simulink model "gm_minutiaeextraction_21821"  (R2018b)
(part 3 of 7)

  t/4845 -> concatenate37/109
  t/4846 -> concatenate37/110
  t/4847 -> concatenate37/111
  t/4848 -> concatenate37/112
  t/4849 -> concatenate37/113
  t/4850 -> concatenate37/114
  t/4851 -> concatenate37/115
  t/4852 -> concatenate37/116
  t/4853 -> concatenate37/117
  t/4854 -> concatenate37/118
  t/4855 -> concatenate37/119
  t/4856 -> concatenate37/120
  t/4857 -> concatenate37/121
  t/4858 -> concatenate37/122
  t/4859 -> concatenate37/123
  t/4860 -> concatenate37/124
  t/4861 -> concatenate37/125
  t/4862 -> concatenate37/126
  t/4863 -> concatenate37/127
  t/4864 -> concatenate37/128
  t/4865 -> concatenate38/1
  t/4866 -> concatenate38/2
  t/4867 -> concatenate38/3
  t/4868 -> concatenate38/4
  t/4869 -> concatenate38/5
  t/4870 -> concatenate38/6
  t/4871 -> concatenate38/7
  t/4872 -> concatenate38/8
  t/4873 -> concatenate38/9
  t/4874 -> concatenate38/10
  t/4875 -> concatenate38/11
  t/4876 -> concatenate38/12
  t/4877 -> concatenate38/13
  t/4878 -> concatenate38/14
  t/4879 -> concatenate38/15
  t/4880 -> concatenate38/16
  t/4881 -> concatenate38/17
  t/4882 -> concatenate38/18
  t/4883 -> concatenate38/19
  t/4884 -> concatenate38/20
  t/4885 -> concatenate38/21
  t/4886 -> concatenate38/22
  t/4887 -> concatenate38/23
  t/4888 -> concatenate38/24
  t/4889 -> concatenate38/25
  t/4890 -> concatenate38/26
  t/4891 -> concatenate38/27
  t/4892 -> concatenate38/28
  t/4893 -> concatenate38/29
  t/4894 -> concatenate38/30
  t/4895 -> concatenate38/31
  t/4896 -> concatenate38/32
  t/4897 -> concatenate38/33
  t/4898 -> concatenate38/34
  t/4899 -> concatenate38/35
  t/4900 -> concatenate38/36
  t/4901 -> concatenate38/37
  t/4902 -> concatenate38/38
  t/4903 -> concatenate38/39
  t/4904 -> concatenate38/40
  t/4905 -> concatenate38/41
  t/4906 -> concatenate38/42
  t/4907 -> concatenate38/43
  t/4908 -> concatenate38/44
  t/4909 -> concatenate38/45
  t/4910 -> concatenate38/46
  t/4911 -> concatenate38/47
  t/4912 -> concatenate38/48
  t/4913 -> concatenate38/49
  t/4914 -> concatenate38/50
  t/4915 -> concatenate38/51
  t/4916 -> concatenate38/52
  t/4917 -> concatenate38/53
  t/4918 -> concatenate38/54
  t/4919 -> concatenate38/55
  t/4920 -> concatenate38/56
  t/4921 -> concatenate38/57
  t/4922 -> concatenate38/58
  t/4923 -> concatenate38/59
  t/4924 -> concatenate38/60
  t/4925 -> concatenate38/61
  t/4926 -> concatenate38/62
  t/4927 -> concatenate38/63
  t/4928 -> concatenate38/64
  t/4929 -> concatenate38/65
  t/4930 -> concatenate38/66
  t/4931 -> concatenate38/67
  t/4932 -> concatenate38/68
  t/4933 -> concatenate38/69
  t/4934 -> concatenate38/70
  t/4935 -> concatenate38/71
  t/4936 -> concatenate38/72
  t/4937 -> concatenate38/73
  t/4938 -> concatenate38/74
  t/4939 -> concatenate38/75
  t/4940 -> concatenate38/76
  t/4941 -> concatenate38/77
  t/4942 -> concatenate38/78
  t/4943 -> concatenate38/79
  t/4944 -> concatenate38/80
  t/4945 -> concatenate38/81
  t/4946 -> concatenate38/82
  t/4947 -> concatenate38/83
  t/4948 -> concatenate38/84
  t/4949 -> concatenate38/85
  t/4950 -> concatenate38/86
  t/4951 -> concatenate38/87
  t/4952 -> concatenate38/88
  t/4953 -> concatenate38/89
  t/4954 -> concatenate38/90
  t/4955 -> concatenate38/91
  t/4956 -> concatenate38/92
  t/4957 -> concatenate38/93
  t/4958 -> concatenate38/94
  t/4959 -> concatenate38/95
  t/4960 -> concatenate38/96
  t/4961 -> concatenate38/97
  t/4962 -> concatenate38/98
  t/4963 -> concatenate38/99
  t/4964 -> concatenate38/100
  t/4965 -> concatenate38/101
  t/4966 -> concatenate38/102
  t/4967 -> concatenate38/103
  t/4968 -> concatenate38/104
  t/4969 -> concatenate38/105
  t/4970 -> concatenate38/106
  t/4971 -> concatenate38/107
  t/4972 -> concatenate38/108
  t/4973 -> concatenate38/109
  t/4974 -> concatenate38/110
  t/4975 -> concatenate38/111
  t/4976 -> concatenate38/112
  t/4977 -> concatenate38/113
  t/4978 -> concatenate38/114
  t/4979 -> concatenate38/115
  t/4980 -> concatenate38/116
  t/4981 -> concatenate38/117
  t/4982 -> concatenate38/118
  t/4983 -> concatenate38/119
  t/4984 -> concatenate38/120
  t/4985 -> concatenate38/121
  t/4986 -> concatenate38/122
  t/4987 -> concatenate38/123
  t/4988 -> concatenate38/124
  t/4989 -> concatenate38/125
  t/4990 -> concatenate38/126
  t/4991 -> concatenate38/127
  t/4992 -> concatenate38/128
  t/4993 -> concatenate39/1
  t/4994 -> concatenate39/2
  t/4995 -> concatenate39/3
  t/4996 -> concatenate39/4
  t/4997 -> concatenate39/5
  t/4998 -> concatenate39/6
  t/4999 -> concatenate39/7
  t/5000 -> concatenate39/8
  t/5001 -> concatenate39/9
  t/5002 -> concatenate39/10
  t/5003 -> concatenate39/11
  t/5004 -> concatenate39/12
  t/5005 -> concatenate39/13
  t/5006 -> concatenate39/14
  t/5007 -> concatenate39/15
  t/5008 -> concatenate39/16
  t/5009 -> concatenate39/17
  t/5010 -> concatenate39/18
  t/5011 -> concatenate39/19
  t/5012 -> concatenate39/20
  t/5013 -> concatenate39/21
  t/5014 -> concatenate39/22
  t/5015 -> concatenate39/23
  t/5016 -> concatenate39/24
  t/5017 -> concatenate39/25
  t/5018 -> concatenate39/26
  t/5019 -> concatenate39/27
  t/5020 -> concatenate39/28
  t/5021 -> concatenate39/29
  t/5022 -> concatenate39/30
  t/5023 -> concatenate39/31
  t/5024 -> concatenate39/32
  t/5025 -> concatenate39/33
  t/5026 -> concatenate39/34
  t/5027 -> concatenate39/35
  t/5028 -> concatenate39/36
  t/5029 -> concatenate39/37
  t/5030 -> concatenate39/38
  t/5031 -> concatenate39/39
  t/5032 -> concatenate39/40
  t/5033 -> concatenate39/41
  t/5034 -> concatenate39/42
  t/5035 -> concatenate39/43
  t/5036 -> concatenate39/44
  t/5037 -> concatenate39/45
  t/5038 -> concatenate39/46
  t/5039 -> concatenate39/47
  t/5040 -> concatenate39/48
  t/5041 -> concatenate39/49
  t/5042 -> concatenate39/50
  t/5043 -> concatenate39/51
  t/5044 -> concatenate39/52
  t/5045 -> concatenate39/53
  t/5046 -> concatenate39/54
  t/5047 -> concatenate39/55
  t/5048 -> concatenate39/56
  t/5049 -> concatenate39/57
  t/5050 -> concatenate39/58
  t/5051 -> concatenate39/59
  t/5052 -> concatenate39/60
  t/5053 -> concatenate39/61
  t/5054 -> concatenate39/62
  t/5055 -> concatenate39/63
  t/5056 -> concatenate39/64
  t/5057 -> concatenate39/65
  t/5058 -> concatenate39/66
  t/5059 -> concatenate39/67
  t/5060 -> concatenate39/68
  t/5061 -> concatenate39/69
  t/5062 -> concatenate39/70
  t/5063 -> concatenate39/71
  t/5064 -> concatenate39/72
  t/5065 -> concatenate39/73
  t/5066 -> concatenate39/74
  t/5067 -> concatenate39/75
  t/5068 -> concatenate39/76
  t/5069 -> concatenate39/77
  t/5070 -> concatenate39/78
  t/5071 -> concatenate39/79
  t/5072 -> concatenate39/80
  t/5073 -> concatenate39/81
  t/5074 -> concatenate39/82
  t/5075 -> concatenate39/83
  t/5076 -> concatenate39/84
  t/5077 -> concatenate39/85
  t/5078 -> concatenate39/86
  t/5079 -> concatenate39/87
  t/5080 -> concatenate39/88
  t/5081 -> concatenate39/89
  t/5082 -> concatenate39/90
  t/5083 -> concatenate39/91
  t/5084 -> concatenate39/92
  t/5085 -> concatenate39/93
  t/5086 -> concatenate39/94
  t/5087 -> concatenate39/95
  t/5088 -> concatenate39/96
  t/5089 -> concatenate39/97
  t/5090 -> concatenate39/98
  t/5091 -> concatenate39/99
  t/5092 -> concatenate39/100
  t/5093 -> concatenate39/101
  t/5094 -> concatenate39/102
  t/5095 -> concatenate39/103
  t/5096 -> concatenate39/104
  t/5097 -> concatenate39/105
  t/5098 -> concatenate39/106
  t/5099 -> concatenate39/107
  t/5100 -> concatenate39/108
  t/5101 -> concatenate39/109
  t/5102 -> concatenate39/110
  t/5103 -> concatenate39/111
  t/5104 -> concatenate39/112
  t/5105 -> concatenate39/113
  t/5106 -> concatenate39/114
  t/5107 -> concatenate39/115
  t/5108 -> concatenate39/116
  t/5109 -> concatenate39/117
  t/5110 -> concatenate39/118
  t/5111 -> concatenate39/119
  t/5112 -> concatenate39/120
  t/5113 -> concatenate39/121
  t/5114 -> concatenate39/122
  t/5115 -> concatenate39/123
  t/5116 -> concatenate39/124
  t/5117 -> concatenate39/125
  t/5118 -> concatenate39/126
  t/5119 -> concatenate39/127
  t/5120 -> concatenate39/128
  t/5121 -> concatenate40/1
  t/5122 -> concatenate40/2
  t/5123 -> concatenate40/3
  t/5124 -> concatenate40/4
  t/5125 -> concatenate40/5
  t/5126 -> concatenate40/6
  t/5127 -> concatenate40/7
  t/5128 -> concatenate40/8
  t/5129 -> concatenate40/9
  t/5130 -> concatenate40/10
  t/5131 -> concatenate40/11
  t/5132 -> concatenate40/12
  t/5133 -> concatenate40/13
  t/5134 -> concatenate40/14
  t/5135 -> concatenate40/15
  t/5136 -> concatenate40/16
  t/5137 -> concatenate40/17
  t/5138 -> concatenate40/18
  t/5139 -> concatenate40/19
  t/5140 -> concatenate40/20
  t/5141 -> concatenate40/21
  t/5142 -> concatenate40/22
  t/5143 -> concatenate40/23
  t/5144 -> concatenate40/24
  t/5145 -> concatenate40/25
  t/5146 -> concatenate40/26
  t/5147 -> concatenate40/27
  t/5148 -> concatenate40/28
  t/5149 -> concatenate40/29
  t/5150 -> concatenate40/30
  t/5151 -> concatenate40/31
  t/5152 -> concatenate40/32
  t/5153 -> concatenate40/33
  t/5154 -> concatenate40/34
  t/5155 -> concatenate40/35
  t/5156 -> concatenate40/36
  t/5157 -> concatenate40/37
  t/5158 -> concatenate40/38
  t/5159 -> concatenate40/39
  t/5160 -> concatenate40/40
  t/5161 -> concatenate40/41
  t/5162 -> concatenate40/42
  t/5163 -> concatenate40/43
  t/5164 -> concatenate40/44
  t/5165 -> concatenate40/45
  t/5166 -> concatenate40/46
  t/5167 -> concatenate40/47
  t/5168 -> concatenate40/48
  t/5169 -> concatenate40/49
  t/5170 -> concatenate40/50
  t/5171 -> concatenate40/51
  t/5172 -> concatenate40/52
  t/5173 -> concatenate40/53
  t/5174 -> concatenate40/54
  t/5175 -> concatenate40/55
  t/5176 -> concatenate40/56
  t/5177 -> concatenate40/57
  t/5178 -> concatenate40/58
  t/5179 -> concatenate40/59
  t/5180 -> concatenate40/60
  t/5181 -> concatenate40/61
  t/5182 -> concatenate40/62
  t/5183 -> concatenate40/63
  t/5184 -> concatenate40/64
  t/5185 -> concatenate40/65
  t/5186 -> concatenate40/66
  t/5187 -> concatenate40/67
  t/5188 -> concatenate40/68
  t/5189 -> concatenate40/69
  t/5190 -> concatenate40/70
  t/5191 -> concatenate40/71
  t/5192 -> concatenate40/72
  t/5193 -> concatenate40/73
  t/5194 -> concatenate40/74
  t/5195 -> concatenate40/75
  t/5196 -> concatenate40/76
  t/5197 -> concatenate40/77
  t/5198 -> concatenate40/78
  t/5199 -> concatenate40/79
  t/5200 -> concatenate40/80
  t/5201 -> concatenate40/81
  t/5202 -> concatenate40/82
  t/5203 -> concatenate40/83
  t/5204 -> concatenate40/84
  t/5205 -> concatenate40/85
  t/5206 -> concatenate40/86
  t/5207 -> concatenate40/87
  t/5208 -> concatenate40/88
  t/5209 -> concatenate40/89
  t/5210 -> concatenate40/90
  t/5211 -> concatenate40/91
  t/5212 -> concatenate40/92
  t/5213 -> concatenate40/93
  t/5214 -> concatenate40/94
  t/5215 -> concatenate40/95
  t/5216 -> concatenate40/96
  t/5217 -> concatenate40/97
  t/5218 -> concatenate40/98
  t/5219 -> concatenate40/99
  t/5220 -> concatenate40/100
  t/5221 -> concatenate40/101
  t/5222 -> concatenate40/102
  t/5223 -> concatenate40/103
  t/5224 -> concatenate40/104
  t/5225 -> concatenate40/105
  t/5226 -> concatenate40/106
  t/5227 -> concatenate40/107
  t/5228 -> concatenate40/108
  t/5229 -> concatenate40/109
  t/5230 -> concatenate40/110
  t/5231 -> concatenate40/111
  t/5232 -> concatenate40/112
  t/5233 -> concatenate40/113
  t/5234 -> concatenate40/114
  t/5235 -> concatenate40/115
  t/5236 -> concatenate40/116
  t/5237 -> concatenate40/117
  t/5238 -> concatenate40/118
  t/5239 -> concatenate40/119
  t/5240 -> concatenate40/120
  t/5241 -> concatenate40/121
  t/5242 -> concatenate40/122
  t/5243 -> concatenate40/123
  t/5244 -> concatenate40/124
  t/5245 -> concatenate40/125
  t/5246 -> concatenate40/126
  t/5247 -> concatenate40/127
  t/5248 -> concatenate40/128
  t/5249 -> concatenate41/1
  t/5250 -> concatenate41/2
  t/5251 -> concatenate41/3
  t/5252 -> concatenate41/4
  t/5253 -> concatenate41/5
  t/5254 -> concatenate41/6
  t/5255 -> concatenate41/7
  t/5256 -> concatenate41/8
  t/5257 -> concatenate41/9
  t/5258 -> concatenate41/10
  t/5259 -> concatenate41/11
  t/5260 -> concatenate41/12
  t/5261 -> concatenate41/13
  t/5262 -> concatenate41/14
  t/5263 -> concatenate41/15
  t/5264 -> concatenate41/16
  t/5265 -> concatenate41/17
  t/5266 -> concatenate41/18
  t/5267 -> concatenate41/19
  t/5268 -> concatenate41/20
  t/5269 -> concatenate41/21
  t/5270 -> concatenate41/22
  t/5271 -> concatenate41/23
  t/5272 -> concatenate41/24
  t/5273 -> concatenate41/25
  t/5274 -> concatenate41/26
  t/5275 -> concatenate41/27
  t/5276 -> concatenate41/28
  t/5277 -> concatenate41/29
  t/5278 -> concatenate41/30
  t/5279 -> concatenate41/31
  t/5280 -> concatenate41/32
  t/5281 -> concatenate41/33
  t/5282 -> concatenate41/34
  t/5283 -> concatenate41/35
  t/5284 -> concatenate41/36
  t/5285 -> concatenate41/37
  t/5286 -> concatenate41/38
  t/5287 -> concatenate41/39
  t/5288 -> concatenate41/40
  t/5289 -> concatenate41/41
  t/5290 -> concatenate41/42
  t/5291 -> concatenate41/43
  t/5292 -> concatenate41/44
  t/5293 -> concatenate41/45
  t/5294 -> concatenate41/46
  t/5295 -> concatenate41/47
  t/5296 -> concatenate41/48
  t/5297 -> concatenate41/49
  t/5298 -> concatenate41/50
  t/5299 -> concatenate41/51
  t/5300 -> concatenate41/52
  t/5301 -> concatenate41/53
  t/5302 -> concatenate41/54
  t/5303 -> concatenate41/55
  t/5304 -> concatenate41/56
  t/5305 -> concatenate41/57
  t/5306 -> concatenate41/58
  t/5307 -> concatenate41/59
  t/5308 -> concatenate41/60
  t/5309 -> concatenate41/61
  t/5310 -> concatenate41/62
  t/5311 -> concatenate41/63
  t/5312 -> concatenate41/64
  t/5313 -> concatenate41/65
  t/5314 -> concatenate41/66
  t/5315 -> concatenate41/67
  t/5316 -> concatenate41/68
  t/5317 -> concatenate41/69
  t/5318 -> concatenate41/70
  t/5319 -> concatenate41/71
  t/5320 -> concatenate41/72
  t/5321 -> concatenate41/73
  t/5322 -> concatenate41/74
  t/5323 -> concatenate41/75
  t/5324 -> concatenate41/76
  t/5325 -> concatenate41/77
  t/5326 -> concatenate41/78
  t/5327 -> concatenate41/79
  t/5328 -> concatenate41/80
  t/5329 -> concatenate41/81
  t/5330 -> concatenate41/82
  t/5331 -> concatenate41/83
  t/5332 -> concatenate41/84
  t/5333 -> concatenate41/85
  t/5334 -> concatenate41/86
  t/5335 -> concatenate41/87
  t/5336 -> concatenate41/88
  t/5337 -> concatenate41/89
  t/5338 -> concatenate41/90
  t/5339 -> concatenate41/91
  t/5340 -> concatenate41/92
  t/5341 -> concatenate41/93
  t/5342 -> concatenate41/94
  t/5343 -> concatenate41/95
  t/5344 -> concatenate41/96
  t/5345 -> concatenate41/97
  t/5346 -> concatenate41/98
  t/5347 -> concatenate41/99
  t/5348 -> concatenate41/100
  t/5349 -> concatenate41/101
  t/5350 -> concatenate41/102
  t/5351 -> concatenate41/103
  t/5352 -> concatenate41/104
  t/5353 -> concatenate41/105
  t/5354 -> concatenate41/106
  t/5355 -> concatenate41/107
  t/5356 -> concatenate41/108
  t/5357 -> concatenate41/109
  t/5358 -> concatenate41/110
  t/5359 -> concatenate41/111
  t/5360 -> concatenate41/112
  t/5361 -> concatenate41/113
  t/5362 -> concatenate41/114
  t/5363 -> concatenate41/115
  t/5364 -> concatenate41/116
  t/5365 -> concatenate41/117
  t/5366 -> concatenate41/118
  t/5367 -> concatenate41/119
  t/5368 -> concatenate41/120
  t/5369 -> concatenate41/121
  t/5370 -> concatenate41/122
  t/5371 -> concatenate41/123
  t/5372 -> concatenate41/124
  t/5373 -> concatenate41/125
  t/5374 -> concatenate41/126
  t/5375 -> concatenate41/127
  t/5376 -> concatenate41/128
  t/5377 -> concatenate42/1
  t/5378 -> concatenate42/2
  t/5379 -> concatenate42/3
  t/5380 -> concatenate42/4
  t/5381 -> concatenate42/5
  t/5382 -> concatenate42/6
  t/5383 -> concatenate42/7
  t/5384 -> concatenate42/8
  t/5385 -> concatenate42/9
  t/5386 -> concatenate42/10
  t/5387 -> concatenate42/11
  t/5388 -> concatenate42/12
  t/5389 -> concatenate42/13
  t/5390 -> concatenate42/14
  t/5391 -> concatenate42/15
  t/5392 -> concatenate42/16
  t/5393 -> concatenate42/17
  t/5394 -> concatenate42/18
  t/5395 -> concatenate42/19
  t/5396 -> concatenate42/20
  t/5397 -> concatenate42/21
  t/5398 -> concatenate42/22
  t/5399 -> concatenate42/23
  t/5400 -> concatenate42/24
  t/5401 -> concatenate42/25
  t/5402 -> concatenate42/26
  t/5403 -> concatenate42/27
  t/5404 -> concatenate42/28
  t/5405 -> concatenate42/29
  t/5406 -> concatenate42/30
  t/5407 -> concatenate42/31
  t/5408 -> concatenate42/32
  t/5409 -> concatenate42/33
  t/5410 -> concatenate42/34
  t/5411 -> concatenate42/35
  t/5412 -> concatenate42/36
  t/5413 -> concatenate42/37
  t/5414 -> concatenate42/38
  t/5415 -> concatenate42/39
  t/5416 -> concatenate42/40
  t/5417 -> concatenate42/41
  t/5418 -> concatenate42/42
  t/5419 -> concatenate42/43
  t/5420 -> concatenate42/44
  t/5421 -> concatenate42/45
  t/5422 -> concatenate42/46
  t/5423 -> concatenate42/47
  t/5424 -> concatenate42/48
  t/5425 -> concatenate42/49
  t/5426 -> concatenate42/50
  t/5427 -> concatenate42/51
  t/5428 -> concatenate42/52
  t/5429 -> concatenate42/53
  t/5430 -> concatenate42/54
  t/5431 -> concatenate42/55
  t/5432 -> concatenate42/56
  t/5433 -> concatenate42/57
  t/5434 -> concatenate42/58
  t/5435 -> concatenate42/59
  t/5436 -> concatenate42/60
  t/5437 -> concatenate42/61
  t/5438 -> concatenate42/62
  t/5439 -> concatenate42/63
  t/5440 -> concatenate42/64
  t/5441 -> concatenate42/65
  t/5442 -> concatenate42/66
  t/5443 -> concatenate42/67
  t/5444 -> concatenate42/68
  t/5445 -> concatenate42/69
  t/5446 -> concatenate42/70
  t/5447 -> concatenate42/71
  t/5448 -> concatenate42/72
  t/5449 -> concatenate42/73
  t/5450 -> concatenate42/74
  t/5451 -> concatenate42/75
  t/5452 -> concatenate42/76
  t/5453 -> concatenate42/77
  t/5454 -> concatenate42/78
  t/5455 -> concatenate42/79
  t/5456 -> concatenate42/80
  t/5457 -> concatenate42/81
  t/5458 -> concatenate42/82
  t/5459 -> concatenate42/83
  t/5460 -> concatenate42/84
  t/5461 -> concatenate42/85
  t/5462 -> concatenate42/86
  t/5463 -> concatenate42/87
  t/5464 -> concatenate42/88
  t/5465 -> concatenate42/89
  t/5466 -> concatenate42/90
  t/5467 -> concatenate42/91
  t/5468 -> concatenate42/92
  t/5469 -> concatenate42/93
  t/5470 -> concatenate42/94
  t/5471 -> concatenate42/95
  t/5472 -> concatenate42/96
  t/5473 -> concatenate42/97
  t/5474 -> concatenate42/98
  t/5475 -> concatenate42/99
  t/5476 -> concatenate42/100
  t/5477 -> concatenate42/101
  t/5478 -> concatenate42/102
  t/5479 -> concatenate42/103
  t/5480 -> concatenate42/104
  t/5481 -> concatenate42/105
  t/5482 -> concatenate42/106
  t/5483 -> concatenate42/107
  t/5484 -> concatenate42/108
  t/5485 -> concatenate42/109
  t/5486 -> concatenate42/110
  t/5487 -> concatenate42/111
  t/5488 -> concatenate42/112
  t/5489 -> concatenate42/113
  t/5490 -> concatenate42/114
  t/5491 -> concatenate42/115
  t/5492 -> concatenate42/116
  t/5493 -> concatenate42/117
  t/5494 -> concatenate42/118
  t/5495 -> concatenate42/119
  t/5496 -> concatenate42/120
  t/5497 -> concatenate42/121
  t/5498 -> concatenate42/122
  t/5499 -> concatenate42/123
  t/5500 -> concatenate42/124
  t/5501 -> concatenate42/125
  t/5502 -> concatenate42/126
  t/5503 -> concatenate42/127
  t/5504 -> concatenate42/128
  t/5505 -> concatenate43/1
  t/5506 -> concatenate43/2
  t/5507 -> concatenate43/3
  t/5508 -> concatenate43/4
  t/5509 -> concatenate43/5
  t/5510 -> concatenate43/6
  t/5511 -> concatenate43/7
  t/5512 -> concatenate43/8
  t/5513 -> concatenate43/9
  t/5514 -> concatenate43/10
  t/5515 -> concatenate43/11
  t/5516 -> concatenate43/12
  t/5517 -> concatenate43/13
  t/5518 -> concatenate43/14
  t/5519 -> concatenate43/15
  t/5520 -> concatenate43/16
  t/5521 -> concatenate43/17
  t/5522 -> concatenate43/18
  t/5523 -> concatenate43/19
  t/5524 -> concatenate43/20
  t/5525 -> concatenate43/21
  t/5526 -> concatenate43/22
  t/5527 -> concatenate43/23
  t/5528 -> concatenate43/24
  t/5529 -> concatenate43/25
  t/5530 -> concatenate43/26
  t/5531 -> concatenate43/27
  t/5532 -> concatenate43/28
  t/5533 -> concatenate43/29
  t/5534 -> concatenate43/30
  t/5535 -> concatenate43/31
  t/5536 -> concatenate43/32
  t/5537 -> concatenate43/33
  t/5538 -> concatenate43/34
  t/5539 -> concatenate43/35
  t/5540 -> concatenate43/36
  t/5541 -> concatenate43/37
  t/5542 -> concatenate43/38
  t/5543 -> concatenate43/39
  t/5544 -> concatenate43/40
  t/5545 -> concatenate43/41
  t/5546 -> concatenate43/42
  t/5547 -> concatenate43/43
  t/5548 -> concatenate43/44
  t/5549 -> concatenate43/45
  t/5550 -> concatenate43/46
  t/5551 -> concatenate43/47
  t/5552 -> concatenate43/48
  t/5553 -> concatenate43/49
  t/5554 -> concatenate43/50
  t/5555 -> concatenate43/51
  t/5556 -> concatenate43/52
  t/5557 -> concatenate43/53
  t/5558 -> concatenate43/54
  t/5559 -> concatenate43/55
  t/5560 -> concatenate43/56
  t/5561 -> concatenate43/57
  t/5562 -> concatenate43/58
  t/5563 -> concatenate43/59
  t/5564 -> concatenate43/60
  t/5565 -> concatenate43/61
  t/5566 -> concatenate43/62
  t/5567 -> concatenate43/63
  t/5568 -> concatenate43/64
  t/5569 -> concatenate43/65
  t/5570 -> concatenate43/66
  t/5571 -> concatenate43/67
  t/5572 -> concatenate43/68
  t/5573 -> concatenate43/69
  t/5574 -> concatenate43/70
  t/5575 -> concatenate43/71
  t/5576 -> concatenate43/72
  t/5577 -> concatenate43/73
  t/5578 -> concatenate43/74
  t/5579 -> concatenate43/75
  t/5580 -> concatenate43/76
  t/5581 -> concatenate43/77
  t/5582 -> concatenate43/78
  t/5583 -> concatenate43/79
  t/5584 -> concatenate43/80
  t/5585 -> concatenate43/81
  t/5586 -> concatenate43/82
  t/5587 -> concatenate43/83
  t/5588 -> concatenate43/84
  t/5589 -> concatenate43/85
  t/5590 -> concatenate43/86
  t/5591 -> concatenate43/87
  t/5592 -> concatenate43/88
  t/5593 -> concatenate43/89
  t/5594 -> concatenate43/90
  t/5595 -> concatenate43/91
  t/5596 -> concatenate43/92
  t/5597 -> concatenate43/93
  t/5598 -> concatenate43/94
  t/5599 -> concatenate43/95
  t/5600 -> concatenate43/96
  t/5601 -> concatenate43/97
  t/5602 -> concatenate43/98
  t/5603 -> concatenate43/99
  t/5604 -> concatenate43/100
  t/5605 -> concatenate43/101
  t/5606 -> concatenate43/102
  t/5607 -> concatenate43/103
  t/5608 -> concatenate43/104
  t/5609 -> concatenate43/105
  t/5610 -> concatenate43/106
  t/5611 -> concatenate43/107
  t/5612 -> concatenate43/108
  t/5613 -> concatenate43/109
  t/5614 -> concatenate43/110
  t/5615 -> concatenate43/111
  t/5616 -> concatenate43/112
  t/5617 -> concatenate43/113
  t/5618 -> concatenate43/114
  t/5619 -> concatenate43/115
  t/5620 -> concatenate43/116
  t/5621 -> concatenate43/117
  t/5622 -> concatenate43/118
  t/5623 -> concatenate43/119
  t/5624 -> concatenate43/120
  t/5625 -> concatenate43/121
  t/5626 -> concatenate43/122
  t/5627 -> concatenate43/123
  t/5628 -> concatenate43/124
  t/5629 -> concatenate43/125
  t/5630 -> concatenate43/126
  t/5631 -> concatenate43/127
  t/5632 -> concatenate43/128
  t/5633 -> concatenate44/1
  t/5634 -> concatenate44/2
  t/5635 -> concatenate44/3
  t/5636 -> concatenate44/4
  t/5637 -> concatenate44/5
  t/5638 -> concatenate44/6
  t/5639 -> concatenate44/7
  t/5640 -> concatenate44/8
  t/5641 -> concatenate44/9
  t/5642 -> concatenate44/10
  t/5643 -> concatenate44/11
  t/5644 -> concatenate44/12
  t/5645 -> concatenate44/13
  t/5646 -> concatenate44/14
  t/5647 -> concatenate44/15
  t/5648 -> concatenate44/16
  t/5649 -> concatenate44/17
  t/5650 -> concatenate44/18
  t/5651 -> concatenate44/19
  t/5652 -> concatenate44/20
  t/5653 -> concatenate44/21
  t/5654 -> concatenate44/22
  t/5655 -> concatenate44/23
  t/5656 -> concatenate44/24
  t/5657 -> concatenate44/25
  t/5658 -> concatenate44/26
  t/5659 -> concatenate44/27
  t/5660 -> concatenate44/28
  t/5661 -> concatenate44/29
  t/5662 -> concatenate44/30
  t/5663 -> concatenate44/31
  t/5664 -> concatenate44/32
  t/5665 -> concatenate44/33
  t/5666 -> concatenate44/34
  t/5667 -> concatenate44/35
  t/5668 -> concatenate44/36
  t/5669 -> concatenate44/37
  t/5670 -> concatenate44/38
  t/5671 -> concatenate44/39
  t/5672 -> concatenate44/40
  t/5673 -> concatenate44/41
  t/5674 -> concatenate44/42
  t/5675 -> concatenate44/43
  t/5676 -> concatenate44/44
  t/5677 -> concatenate44/45
  t/5678 -> concatenate44/46
  t/5679 -> concatenate44/47
  t/5680 -> concatenate44/48
  t/5681 -> concatenate44/49
  t/5682 -> concatenate44/50
  t/5683 -> concatenate44/51
  t/5684 -> concatenate44/52
  t/5685 -> concatenate44/53
  t/5686 -> concatenate44/54
  t/5687 -> concatenate44/55
  t/5688 -> concatenate44/56
  t/5689 -> concatenate44/57
  t/5690 -> concatenate44/58
  t/5691 -> concatenate44/59
  t/5692 -> concatenate44/60
  t/5693 -> concatenate44/61
  t/5694 -> concatenate44/62
  t/5695 -> concatenate44/63
  t/5696 -> concatenate44/64
  t/5697 -> concatenate44/65
  t/5698 -> concatenate44/66
  t/5699 -> concatenate44/67
  t/5700 -> concatenate44/68
  t/5701 -> concatenate44/69
  t/5702 -> concatenate44/70
  t/5703 -> concatenate44/71
  t/5704 -> concatenate44/72
  t/5705 -> concatenate44/73
  t/5706 -> concatenate44/74
  t/5707 -> concatenate44/75
  t/5708 -> concatenate44/76
  t/5709 -> concatenate44/77
  t/5710 -> concatenate44/78
  t/5711 -> concatenate44/79
  t/5712 -> concatenate44/80
  t/5713 -> concatenate44/81
  t/5714 -> concatenate44/82
  t/5715 -> concatenate44/83
  t/5716 -> concatenate44/84
  t/5717 -> concatenate44/85
  t/5718 -> concatenate44/86
  t/5719 -> concatenate44/87
  t/5720 -> concatenate44/88
  t/5721 -> concatenate44/89
  t/5722 -> concatenate44/90
  t/5723 -> concatenate44/91
  t/5724 -> concatenate44/92
  t/5725 -> concatenate44/93
  t/5726 -> concatenate44/94
  t/5727 -> concatenate44/95
  t/5728 -> concatenate44/96
  t/5729 -> concatenate44/97
  t/5730 -> concatenate44/98
  t/5731 -> concatenate44/99
  t/5732 -> concatenate44/100
  t/5733 -> concatenate44/101
  t/5734 -> concatenate44/102
  t/5735 -> concatenate44/103
  t/5736 -> concatenate44/104
  t/5737 -> concatenate44/105
  t/5738 -> concatenate44/106
  t/5739 -> concatenate44/107
  t/5740 -> concatenate44/108
  t/5741 -> concatenate44/109
  t/5742 -> concatenate44/110
  t/5743 -> concatenate44/111
  t/5744 -> concatenate44/112
  t/5745 -> concatenate44/113
  t/5746 -> concatenate44/114
  t/5747 -> concatenate44/115
  t/5748 -> concatenate44/116
  t/5749 -> concatenate44/117
  t/5750 -> concatenate44/118
  t/5751 -> concatenate44/119
  t/5752 -> concatenate44/120
  t/5753 -> concatenate44/121
  t/5754 -> concatenate44/122
  t/5755 -> concatenate44/123
  t/5756 -> concatenate44/124
  t/5757 -> concatenate44/125
  t/5758 -> concatenate44/126
  t/5759 -> concatenate44/127
  t/5760 -> concatenate44/128
  t/5761 -> concatenate45/1
  t/5762 -> concatenate45/2
  t/5763 -> concatenate45/3
  t/5764 -> concatenate45/4
  t/5765 -> concatenate45/5
  t/5766 -> concatenate45/6
  t/5767 -> concatenate45/7
  t/5768 -> concatenate45/8
  t/5769 -> concatenate45/9
  t/5770 -> concatenate45/10
  t/5771 -> concatenate45/11
  t/5772 -> concatenate45/12
  t/5773 -> concatenate45/13
  t/5774 -> concatenate45/14
  t/5775 -> concatenate45/15
  t/5776 -> concatenate45/16
  t/5777 -> concatenate45/17
  t/5778 -> concatenate45/18
  t/5779 -> concatenate45/19
  t/5780 -> concatenate45/20
  t/5781 -> concatenate45/21
  t/5782 -> concatenate45/22
  t/5783 -> concatenate45/23
  t/5784 -> concatenate45/24
  t/5785 -> concatenate45/25
  t/5786 -> concatenate45/26
  t/5787 -> concatenate45/27
  t/5788 -> concatenate45/28
  t/5789 -> concatenate45/29
  t/5790 -> concatenate45/30
  t/5791 -> concatenate45/31
  t/5792 -> concatenate45/32
  t/5793 -> concatenate45/33
  t/5794 -> concatenate45/34
  t/5795 -> concatenate45/35
  t/5796 -> concatenate45/36
  t/5797 -> concatenate45/37
  t/5798 -> concatenate45/38
  t/5799 -> concatenate45/39
  t/5800 -> concatenate45/40
  t/5801 -> concatenate45/41
  t/5802 -> concatenate45/42
  t/5803 -> concatenate45/43
  t/5804 -> concatenate45/44
  t/5805 -> concatenate45/45
  t/5806 -> concatenate45/46
  t/5807 -> concatenate45/47
  t/5808 -> concatenate45/48
  t/5809 -> concatenate45/49
  t/5810 -> concatenate45/50
  t/5811 -> concatenate45/51
  t/5812 -> concatenate45/52
  t/5813 -> concatenate45/53
  t/5814 -> concatenate45/54
  t/5815 -> concatenate45/55
  t/5816 -> concatenate45/56
  t/5817 -> concatenate45/57
  t/5818 -> concatenate45/58
  t/5819 -> concatenate45/59
  t/5820 -> concatenate45/60
  t/5821 -> concatenate45/61
  t/5822 -> concatenate45/62
  t/5823 -> concatenate45/63
  t/5824 -> concatenate45/64
  t/5825 -> concatenate45/65
  t/5826 -> concatenate45/66
  t/5827 -> concatenate45/67
  t/5828 -> concatenate45/68
  t/5829 -> concatenate45/69
  t/5830 -> concatenate45/70
  t/5831 -> concatenate45/71
  t/5832 -> concatenate45/72
  t/5833 -> concatenate45/73
  t/5834 -> concatenate45/74
  t/5835 -> concatenate45/75
  t/5836 -> concatenate45/76
  t/5837 -> concatenate45/77
  t/5838 -> concatenate45/78
  t/5839 -> concatenate45/79
  t/5840 -> concatenate45/80
  t/5841 -> concatenate45/81
  t/5842 -> concatenate45/82
  t/5843 -> concatenate45/83
  t/5844 -> concatenate45/84
  t/5845 -> concatenate45/85
  t/5846 -> concatenate45/86
  t/5847 -> concatenate45/87
  t/5848 -> concatenate45/88
  t/5849 -> concatenate45/89
  t/5850 -> concatenate45/90
  t/5851 -> concatenate45/91
  t/5852 -> concatenate45/92
  t/5853 -> concatenate45/93
  t/5854 -> concatenate45/94
  t/5855 -> concatenate45/95
  t/5856 -> concatenate45/96
  t/5857 -> concatenate45/97
  t/5858 -> concatenate45/98
  t/5859 -> concatenate45/99
  t/5860 -> concatenate45/100
  t/5861 -> concatenate45/101
  t/5862 -> concatenate45/102
  t/5863 -> concatenate45/103
  t/5864 -> concatenate45/104
  t/5865 -> concatenate45/105
  t/5866 -> concatenate45/106
  t/5867 -> concatenate45/107
  t/5868 -> concatenate45/108
  t/5869 -> concatenate45/109
  t/5870 -> concatenate45/110
  t/5871 -> concatenate45/111
  t/5872 -> concatenate45/112
  t/5873 -> concatenate45/113
  t/5874 -> concatenate45/114
  t/5875 -> concatenate45/115
  t/5876 -> concatenate45/116
  t/5877 -> concatenate45/117
  t/5878 -> concatenate45/118
  t/5879 -> concatenate45/119
  t/5880 -> concatenate45/120
  t/5881 -> concatenate45/121
  t/5882 -> concatenate45/122
  t/5883 -> concatenate45/123
  t/5884 -> concatenate45/124
  t/5885 -> concatenate45/125
  t/5886 -> concatenate45/126
  t/5887 -> concatenate45/127
  t/5888 -> concatenate45/128
  t/5889 -> concatenate46/1
  t/5890 -> concatenate46/2
  t/5891 -> concatenate46/3
  t/5892 -> concatenate46/4
  t/5893 -> concatenate46/5
  t/5894 -> concatenate46/6
  t/5895 -> concatenate46/7
  t/5896 -> concatenate46/8
  t/5897 -> concatenate46/9
  t/5898 -> concatenate46/10
  t/5899 -> concatenate46/11
  t/5900 -> concatenate46/12
  t/5901 -> concatenate46/13
  t/5902 -> concatenate46/14
  t/5903 -> concatenate46/15
  t/5904 -> concatenate46/16
  t/5905 -> concatenate46/17
  t/5906 -> concatenate46/18
  t/5907 -> concatenate46/19
  t/5908 -> concatenate46/20
  t/5909 -> concatenate46/21
  t/5910 -> concatenate46/22
  t/5911 -> concatenate46/23
  t/5912 -> concatenate46/24
  t/5913 -> concatenate46/25
  t/5914 -> concatenate46/26
  t/5915 -> concatenate46/27
  t/5916 -> concatenate46/28
  t/5917 -> concatenate46/29
  t/5918 -> concatenate46/30
  t/5919 -> concatenate46/31
  t/5920 -> concatenate46/32
  t/5921 -> concatenate46/33
  t/5922 -> concatenate46/34
  t/5923 -> concatenate46/35
  t/5924 -> concatenate46/36
  t/5925 -> concatenate46/37
  t/5926 -> concatenate46/38
  t/5927 -> concatenate46/39
  t/5928 -> concatenate46/40
  t/5929 -> concatenate46/41
  t/5930 -> concatenate46/42
  t/5931 -> concatenate46/43
  t/5932 -> concatenate46/44
  t/5933 -> concatenate46/45
  t/5934 -> concatenate46/46
  t/5935 -> concatenate46/47
  t/5936 -> concatenate46/48
  t/5937 -> concatenate46/49
  t/5938 -> concatenate46/50
  t/5939 -> concatenate46/51
  t/5940 -> concatenate46/52
  t/5941 -> concatenate46/53
  t/5942 -> concatenate46/54
  t/5943 -> concatenate46/55
  t/5944 -> concatenate46/56
  t/5945 -> concatenate46/57
  t/5946 -> concatenate46/58
  t/5947 -> concatenate46/59
  t/5948 -> concatenate46/60
  t/5949 -> concatenate46/61
  t/5950 -> concatenate46/62
  t/5951 -> concatenate46/63
  t/5952 -> concatenate46/64
  t/5953 -> concatenate46/65
  t/5954 -> concatenate46/66
  t/5955 -> concatenate46/67
  t/5956 -> concatenate46/68
  t/5957 -> concatenate46/69
  t/5958 -> concatenate46/70
  t/5959 -> concatenate46/71
  t/5960 -> concatenate46/72
  t/5961 -> concatenate46/73
  t/5962 -> concatenate46/74
  t/5963 -> concatenate46/75
  t/5964 -> concatenate46/76
  t/5965 -> concatenate46/77
  t/5966 -> concatenate46/78
  t/5967 -> concatenate46/79
  t/5968 -> concatenate46/80
  t/5969 -> concatenate46/81
  t/5970 -> concatenate46/82
  t/5971 -> concatenate46/83
  t/5972 -> concatenate46/84
  t/5973 -> concatenate46/85
  t/5974 -> concatenate46/86
  t/5975 -> concatenate46/87
  t/5976 -> concatenate46/88
  t/5977 -> concatenate46/89
  t/5978 -> concatenate46/90
  t/5979 -> concatenate46/91
  t/5980 -> concatenate46/92
  t/5981 -> concatenate46/93
  t/5982 -> concatenate46/94
  t/5983 -> concatenate46/95
  t/5984 -> concatenate46/96
  t/5985 -> concatenate46/97
  t/5986 -> concatenate46/98
  t/5987 -> concatenate46/99
  t/5988 -> concatenate46/100
  t/5989 -> concatenate46/101
  t/5990 -> concatenate46/102
  t/5991 -> concatenate46/103
  t/5992 -> concatenate46/104
  t/5993 -> concatenate46/105
  t/5994 -> concatenate46/106
  t/5995 -> concatenate46/107
  t/5996 -> concatenate46/108
  t/5997 -> concatenate46/109
  t/5998 -> concatenate46/110
  t/5999 -> concatenate46/111
  t/6000 -> concatenate46/112
  t/6001 -> concatenate46/113
  t/6002 -> concatenate46/114
  t/6003 -> concatenate46/115
  t/6004 -> concatenate46/116
  t/6005 -> concatenate46/117
  t/6006 -> concatenate46/118
  t/6007 -> concatenate46/119
  t/6008 -> concatenate46/120
  t/6009 -> concatenate46/121
  t/6010 -> concatenate46/122
  t/6011 -> concatenate46/123
  t/6012 -> concatenate46/124
  t/6013 -> concatenate46/125
  t/6014 -> concatenate46/126
  t/6015 -> concatenate46/127
  t/6016 -> concatenate46/128
  t/6017 -> concatenate47/1
  t/6018 -> concatenate47/2
  t/6019 -> concatenate47/3
  t/6020 -> concatenate47/4
  t/6021 -> concatenate47/5
  t/6022 -> concatenate47/6
  t/6023 -> concatenate47/7
  t/6024 -> concatenate47/8
  t/6025 -> concatenate47/9
  t/6026 -> concatenate47/10
  t/6027 -> concatenate47/11
  t/6028 -> concatenate47/12
  t/6029 -> concatenate47/13
  t/6030 -> concatenate47/14
  t/6031 -> concatenate47/15
  t/6032 -> concatenate47/16
  t/6033 -> concatenate47/17
  t/6034 -> concatenate47/18
  t/6035 -> concatenate47/19
  t/6036 -> concatenate47/20
  t/6037 -> concatenate47/21
  t/6038 -> concatenate47/22
  t/6039 -> concatenate47/23
  t/6040 -> concatenate47/24
  t/6041 -> concatenate47/25
  t/6042 -> concatenate47/26
  t/6043 -> concatenate47/27
  t/6044 -> concatenate47/28
  t/6045 -> concatenate47/29
  t/6046 -> concatenate47/30
  t/6047 -> concatenate47/31
  t/6048 -> concatenate47/32
  t/6049 -> concatenate47/33
  t/6050 -> concatenate47/34
  t/6051 -> concatenate47/35
  t/6052 -> concatenate47/36
  t/6053 -> concatenate47/37
  t/6054 -> concatenate47/38
  t/6055 -> concatenate47/39
  t/6056 -> concatenate47/40
  t/6057 -> concatenate47/41
  t/6058 -> concatenate47/42
  t/6059 -> concatenate47/43
  t/6060 -> concatenate47/44
  t/6061 -> concatenate47/45
  t/6062 -> concatenate47/46
  t/6063 -> concatenate47/47
  t/6064 -> concatenate47/48
  t/6065 -> concatenate47/49
  t/6066 -> concatenate47/50
  t/6067 -> concatenate47/51
  t/6068 -> concatenate47/52
  t/6069 -> concatenate47/53
  t/6070 -> concatenate47/54
  t/6071 -> concatenate47/55
  t/6072 -> concatenate47/56
  t/6073 -> concatenate47/57
  t/6074 -> concatenate47/58
  t/6075 -> concatenate47/59
  t/6076 -> concatenate47/60
  t/6077 -> concatenate47/61
  t/6078 -> concatenate47/62
  t/6079 -> concatenate47/63
  t/6080 -> concatenate47/64
  t/6081 -> concatenate47/65
  t/6082 -> concatenate47/66
  t/6083 -> concatenate47/67
  t/6084 -> concatenate47/68
  t/6085 -> concatenate47/69
  t/6086 -> concatenate47/70
  t/6087 -> concatenate47/71
  t/6088 -> concatenate47/72
  t/6089 -> concatenate47/73
  t/6090 -> concatenate47/74
  t/6091 -> concatenate47/75
  t/6092 -> concatenate47/76
  t/6093 -> concatenate47/77
  t/6094 -> concatenate47/78
  t/6095 -> concatenate47/79
  t/6096 -> concatenate47/80
  t/6097 -> concatenate47/81
  t/6098 -> concatenate47/82
  t/6099 -> concatenate47/83
  t/6100 -> concatenate47/84
  t/6101 -> concatenate47/85
  t/6102 -> concatenate47/86
  t/6103 -> concatenate47/87
  t/6104 -> concatenate47/88
  t/6105 -> concatenate47/89
  t/6106 -> concatenate47/90
  t/6107 -> concatenate47/91
  t/6108 -> concatenate47/92
  t/6109 -> concatenate47/93
  t/6110 -> concatenate47/94
  t/6111 -> concatenate47/95
  t/6112 -> concatenate47/96
  t/6113 -> concatenate47/97
  t/6114 -> concatenate47/98
  t/6115 -> concatenate47/99
  t/6116 -> concatenate47/100
  t/6117 -> concatenate47/101
  t/6118 -> concatenate47/102
  t/6119 -> concatenate47/103
  t/6120 -> concatenate47/104
  t/6121 -> concatenate47/105
  t/6122 -> concatenate47/106
  t/6123 -> concatenate47/107
  t/6124 -> concatenate47/108
  t/6125 -> concatenate47/109
  t/6126 -> concatenate47/110
  t/6127 -> concatenate47/111
  t/6128 -> concatenate47/112
  t/6129 -> concatenate47/113
  t/6130 -> concatenate47/114
  t/6131 -> concatenate47/115
  t/6132 -> concatenate47/116
  t/6133 -> concatenate47/117
  t/6134 -> concatenate47/118
  t/6135 -> concatenate47/119
  t/6136 -> concatenate47/120
  t/6137 -> concatenate47/121
  t/6138 -> concatenate47/122
  t/6139 -> concatenate47/123
  t/6140 -> concatenate47/124
  t/6141 -> concatenate47/125
  t/6142 -> concatenate47/126
  t/6143 -> concatenate47/127
  t/6144 -> concatenate47/128
  t/6145 -> concatenate48/1
  t/6146 -> concatenate48/2
  t/6147 -> concatenate48/3
  t/6148 -> concatenate48/4
  t/6149 -> concatenate48/5
  t/6150 -> concatenate48/6
  t/6151 -> concatenate48/7
  t/6152 -> concatenate48/8
  t/6153 -> concatenate48/9
  t/6154 -> concatenate48/10
  t/6155 -> concatenate48/11
  t/6156 -> concatenate48/12
  t/6157 -> concatenate48/13
  t/6158 -> concatenate48/14
  t/6159 -> concatenate48/15
  t/6160 -> concatenate48/16
  t/6161 -> concatenate48/17
  t/6162 -> concatenate48/18
  t/6163 -> concatenate48/19
  t/6164 -> concatenate48/20
  t/6165 -> concatenate48/21
  t/6166 -> concatenate48/22
  t/6167 -> concatenate48/23
  t/6168 -> concatenate48/24
  t/6169 -> concatenate48/25
  t/6170 -> concatenate48/26
  t/6171 -> concatenate48/27
  t/6172 -> concatenate48/28
  t/6173 -> concatenate48/29
  t/6174 -> concatenate48/30
  t/6175 -> concatenate48/31
  t/6176 -> concatenate48/32
  t/6177 -> concatenate48/33
  t/6178 -> concatenate48/34
  t/6179 -> concatenate48/35
  t/6180 -> concatenate48/36
  t/6181 -> concatenate48/37
  t/6182 -> concatenate48/38
  t/6183 -> concatenate48/39
  t/6184 -> concatenate48/40
  t/6185 -> concatenate48/41
  t/6186 -> concatenate48/42
  t/6187 -> concatenate48/43
  t/6188 -> concatenate48/44
  t/6189 -> concatenate48/45
  t/6190 -> concatenate48/46
  t/6191 -> concatenate48/47
  t/6192 -> concatenate48/48
  t/6193 -> concatenate48/49
  t/6194 -> concatenate48/50
  t/6195 -> concatenate48/51
  t/6196 -> concatenate48/52
  t/6197 -> concatenate48/53
  t/6198 -> concatenate48/54
  t/6199 -> concatenate48/55
  t/6200 -> concatenate48/56
  t/6201 -> concatenate48/57
  t/6202 -> concatenate48/58
  t/6203 -> concatenate48/59
  t/6204 -> concatenate48/60
  t/6205 -> concatenate48/61
  t/6206 -> concatenate48/62
  t/6207 -> concatenate48/63
  t/6208 -> concatenate48/64
  t/6209 -> concatenate48/65
  t/6210 -> concatenate48/66
  t/6211 -> concatenate48/67
  t/6212 -> concatenate48/68
  t/6213 -> concatenate48/69
  t/6214 -> concatenate48/70
  t/6215 -> concatenate48/71
  t/6216 -> concatenate48/72
  t/6217 -> concatenate48/73
  t/6218 -> concatenate48/74
  t/6219 -> concatenate48/75
  t/6220 -> concatenate48/76
  t/6221 -> concatenate48/77
  t/6222 -> concatenate48/78
  t/6223 -> concatenate48/79
  t/6224 -> concatenate48/80
  t/6225 -> concatenate48/81
  t/6226 -> concatenate48/82
  t/6227 -> concatenate48/83
  t/6228 -> concatenate48/84
  t/6229 -> concatenate48/85
  t/6230 -> concatenate48/86
  t/6231 -> concatenate48/87
  t/6232 -> concatenate48/88
  t/6233 -> concatenate48/89
  t/6234 -> concatenate48/90
  t/6235 -> concatenate48/91
  t/6236 -> concatenate48/92
  t/6237 -> concatenate48/93
  t/6238 -> concatenate48/94
  t/6239 -> concatenate48/95
  t/6240 -> concatenate48/96
  t/6241 -> concatenate48/97
  t/6242 -> concatenate48/98
  t/6243 -> concatenate48/99
  t/6244 -> concatenate48/100
  t/6245 -> concatenate48/101
  t/6246 -> concatenate48/102
  t/6247 -> concatenate48/103
  t/6248 -> concatenate48/104
  t/6249 -> concatenate48/105
  t/6250 -> concatenate48/106
  t/6251 -> concatenate48/107
  t/6252 -> concatenate48/108
  t/6253 -> concatenate48/109
  t/6254 -> concatenate48/110
  t/6255 -> concatenate48/111
  t/6256 -> concatenate48/112
  t/6257 -> concatenate48/113
  t/6258 -> concatenate48/114
  t/6259 -> concatenate48/115
  t/6260 -> concatenate48/116
  t/6261 -> concatenate48/117
  t/6262 -> concatenate48/118
  t/6263 -> concatenate48/119
  t/6264 -> concatenate48/120
  t/6265 -> concatenate48/121
  t/6266 -> concatenate48/122
  t/6267 -> concatenate48/123
  t/6268 -> concatenate48/124
  t/6269 -> concatenate48/125
  t/6270 -> concatenate48/126
  t/6271 -> concatenate48/127
  t/6272 -> concatenate48/128
  t/6273 -> concatenate49/1
  t/6274 -> concatenate49/2
  t/6275 -> concatenate49/3
  t/6276 -> concatenate49/4
  t/6277 -> concatenate49/5
  t/6278 -> concatenate49/6
  t/6279 -> concatenate49/7
  t/6280 -> concatenate49/8
  t/6281 -> concatenate49/9
  t/6282 -> concatenate49/10
  t/6283 -> concatenate49/11
  t/6284 -> concatenate49/12
  t/6285 -> concatenate49/13
  t/6286 -> concatenate49/14
  t/6287 -> concatenate49/15
  t/6288 -> concatenate49/16
  t/6289 -> concatenate49/17
  t/6290 -> concatenate49/18
  t/6291 -> concatenate49/19
  t/6292 -> concatenate49/20
  t/6293 -> concatenate49/21
  t/6294 -> concatenate49/22
  t/6295 -> concatenate49/23
  t/6296 -> concatenate49/24
  t/6297 -> concatenate49/25
  t/6298 -> concatenate49/26
  t/6299 -> concatenate49/27
  t/6300 -> concatenate49/28
  t/6301 -> concatenate49/29
  t/6302 -> concatenate49/30
  t/6303 -> concatenate49/31
  t/6304 -> concatenate49/32
  t/6305 -> concatenate49/33
  t/6306 -> concatenate49/34
  t/6307 -> concatenate49/35
  t/6308 -> concatenate49/36
  t/6309 -> concatenate49/37
  t/6310 -> concatenate49/38
  t/6311 -> concatenate49/39
  t/6312 -> concatenate49/40
  t/6313 -> concatenate49/41
  t/6314 -> concatenate49/42
  t/6315 -> concatenate49/43
  t/6316 -> concatenate49/44
  t/6317 -> concatenate49/45
  t/6318 -> concatenate49/46
  t/6319 -> concatenate49/47
  t/6320 -> concatenate49/48
  t/6321 -> concatenate49/49
  t/6322 -> concatenate49/50
  t/6323 -> concatenate49/51
  t/6324 -> concatenate49/52
  t/6325 -> concatenate49/53
  t/6326 -> concatenate49/54
  t/6327 -> concatenate49/55
  t/6328 -> concatenate49/56
  t/6329 -> concatenate49/57
  t/6330 -> concatenate49/58
  t/6331 -> concatenate49/59
  t/6332 -> concatenate49/60
  t/6333 -> concatenate49/61
  t/6334 -> concatenate49/62
  t/6335 -> concatenate49/63
  t/6336 -> concatenate49/64
  t/6337 -> concatenate49/65
  t/6338 -> concatenate49/66
  t/6339 -> concatenate49/67
  t/6340 -> concatenate49/68
  t/6341 -> concatenate49/69
  t/6342 -> concatenate49/70
  t/6343 -> concatenate49/71
  t/6344 -> concatenate49/72
  t/6345 -> concatenate49/73
  t/6346 -> concatenate49/74
  t/6347 -> concatenate49/75
  t/6348 -> concatenate49/76
  t/6349 -> concatenate49/77
  t/6350 -> concatenate49/78
  t/6351 -> concatenate49/79
  t/6352 -> concatenate49/80
  t/6353 -> concatenate49/81
  t/6354 -> concatenate49/82
  t/6355 -> concatenate49/83
  t/6356 -> concatenate49/84
  t/6357 -> concatenate49/85
  t/6358 -> concatenate49/86
  t/6359 -> concatenate49/87
  t/6360 -> concatenate49/88
  t/6361 -> concatenate49/89
  t/6362 -> concatenate49/90
  t/6363 -> concatenate49/91
  t/6364 -> concatenate49/92
  t/6365 -> concatenate49/93
  t/6366 -> concatenate49/94
  t/6367 -> concatenate49/95
  t/6368 -> concatenate49/96
  t/6369 -> concatenate49/97
  t/6370 -> concatenate49/98
  t/6371 -> concatenate49/99
  t/6372 -> concatenate49/100
  t/6373 -> concatenate49/101
  t/6374 -> concatenate49/102
  t/6375 -> concatenate49/103
  t/6376 -> concatenate49/104
  t/6377 -> concatenate49/105
  t/6378 -> concatenate49/106
  t/6379 -> concatenate49/107
  t/6380 -> concatenate49/108
  t/6381 -> concatenate49/109
  t/6382 -> concatenate49/110
  t/6383 -> concatenate49/111
  t/6384 -> concatenate49/112
  t/6385 -> concatenate49/113
  t/6386 -> concatenate49/114
  t/6387 -> concatenate49/115
  t/6388 -> concatenate49/116
  t/6389 -> concatenate49/117
  t/6390 -> concatenate49/118
  t/6391 -> concatenate49/119
  t/6392 -> concatenate49/120
  t/6393 -> concatenate49/121
  t/6394 -> concatenate49/122
  t/6395 -> concatenate49/123
  t/6396 -> concatenate49/124
  t/6397 -> concatenate49/125
  t/6398 -> concatenate49/126
  t/6399 -> concatenate49/127
  t/6400 -> concatenate49/128
  t/6401 -> concatenate50/1
  t/6402 -> concatenate50/2
  t/6403 -> concatenate50/3
  t/6404 -> concatenate50/4
  t/6405 -> concatenate50/5
  t/6406 -> concatenate50/6
  t/6407 -> concatenate50/7
  t/6408 -> concatenate50/8
  t/6409 -> concatenate50/9
  t/6410 -> concatenate50/10
  t/6411 -> concatenate50/11
  t/6412 -> concatenate50/12
  t/6413 -> concatenate50/13
  t/6414 -> concatenate50/14
  t/6415 -> concatenate50/15
  t/6416 -> concatenate50/16
  t/6417 -> concatenate50/17
  t/6418 -> concatenate50/18
  t/6419 -> concatenate50/19
  t/6420 -> concatenate50/20
  t/6421 -> concatenate50/21
  t/6422 -> concatenate50/22
  t/6423 -> concatenate50/23
  t/6424 -> concatenate50/24
  t/6425 -> concatenate50/25
  t/6426 -> concatenate50/26
  t/6427 -> concatenate50/27
  t/6428 -> concatenate50/28
  t/6429 -> concatenate50/29
  t/6430 -> concatenate50/30
  t/6431 -> concatenate50/31
  t/6432 -> concatenate50/32
  t/6433 -> concatenate50/33
  t/6434 -> concatenate50/34
  t/6435 -> concatenate50/35
  t/6436 -> concatenate50/36
  t/6437 -> concatenate50/37
  t/6438 -> concatenate50/38
  t/6439 -> concatenate50/39
  t/6440 -> concatenate50/40
  t/6441 -> concatenate50/41
  t/6442 -> concatenate50/42
  t/6443 -> concatenate50/43
  t/6444 -> concatenate50/44
  t/6445 -> concatenate50/45
  t/6446 -> concatenate50/46
  t/6447 -> concatenate50/47
  t/6448 -> concatenate50/48
  t/6449 -> concatenate50/49
  t/6450 -> concatenate50/50
  t/6451 -> concatenate50/51
  t/6452 -> concatenate50/52
  t/6453 -> concatenate50/53
  t/6454 -> concatenate50/54
  t/6455 -> concatenate50/55
  t/6456 -> concatenate50/56
  t/6457 -> concatenate50/57
  t/6458 -> concatenate50/58
  t/6459 -> concatenate50/59
  t/6460 -> concatenate50/60
  t/6461 -> concatenate50/61
  t/6462 -> concatenate50/62
  t/6463 -> concatenate50/63
  t/6464 -> concatenate50/64
  t/6465 -> concatenate50/65
  t/6466 -> concatenate50/66
  t/6467 -> concatenate50/67
  t/6468 -> concatenate50/68
  t/6469 -> concatenate50/69
  t/6470 -> concatenate50/70
  t/6471 -> concatenate50/71
  t/6472 -> concatenate50/72
  t/6473 -> concatenate50/73
  t/6474 -> concatenate50/74
  t/6475 -> concatenate50/75
  t/6476 -> concatenate50/76
  t/6477 -> concatenate50/77
  t/6478 -> concatenate50/78
  t/6479 -> concatenate50/79
  t/6480 -> concatenate50/80
  t/6481 -> concatenate50/81
  t/6482 -> concatenate50/82
  t/6483 -> concatenate50/83
  t/6484 -> concatenate50/84
  t/6485 -> concatenate50/85
  t/6486 -> concatenate50/86
  t/6487 -> concatenate50/87
  t/6488 -> concatenate50/88
  t/6489 -> concatenate50/89
  t/6490 -> concatenate50/90
  t/6491 -> concatenate50/91
  t/6492 -> concatenate50/92
  t/6493 -> concatenate50/93
  t/6494 -> concatenate50/94
  t/6495 -> concatenate50/95
  t/6496 -> concatenate50/96
  t/6497 -> concatenate50/97
  t/6498 -> concatenate50/98
  t/6499 -> concatenate50/99
  t/6500 -> concatenate50/100
  t/6501 -> concatenate50/101
  t/6502 -> concatenate50/102
  t/6503 -> concatenate50/103
  t/6504 -> concatenate50/104
  t/6505 -> concatenate50/105
  t/6506 -> concatenate50/106
  t/6507 -> concatenate50/107
  t/6508 -> concatenate50/108
  t/6509 -> concatenate50/109
  t/6510 -> concatenate50/110
  t/6511 -> concatenate50/111
  t/6512 -> concatenate50/112
  t/6513 -> concatenate50/113
  t/6514 -> concatenate50/114
  t/6515 -> concatenate50/115
  t/6516 -> concatenate50/116
  t/6517 -> concatenate50/117
  t/6518 -> concatenate50/118
  t/6519 -> concatenate50/119
  t/6520 -> concatenate50/120
  t/6521 -> concatenate50/121
  t/6522 -> concatenate50/122
  t/6523 -> concatenate50/123
  t/6524 -> concatenate50/124
  t/6525 -> concatenate50/125
  t/6526 -> concatenate50/126
  t/6527 -> concatenate50/127
  t/6528 -> concatenate50/128
  t/6529 -> concatenate51/1
  t/6530 -> concatenate51/2
  t/6531 -> concatenate51/3
  t/6532 -> concatenate51/4
  t/6533 -> concatenate51/5
  t/6534 -> concatenate51/6
  t/6535 -> concatenate51/7
  t/6536 -> concatenate51/8
  t/6537 -> concatenate51/9
  t/6538 -> concatenate51/10
  t/6539 -> concatenate51/11
  t/6540 -> concatenate51/12
  t/6541 -> concatenate51/13
  t/6542 -> concatenate51/14
  t/6543 -> concatenate51/15
  t/6544 -> concatenate51/16
  t/6545 -> concatenate51/17
  t/6546 -> concatenate51/18
  t/6547 -> concatenate51/19
  t/6548 -> concatenate51/20
  t/6549 -> concatenate51/21
  t/6550 -> concatenate51/22
  t/6551 -> concatenate51/23
  t/6552 -> concatenate51/24
  t/6553 -> concatenate51/25
  t/6554 -> concatenate51/26
  t/6555 -> concatenate51/27
  t/6556 -> concatenate51/28
  t/6557 -> concatenate51/29
  t/6558 -> concatenate51/30
  t/6559 -> concatenate51/31
  t/6560 -> concatenate51/32
  t/6561 -> concatenate51/33
  t/6562 -> concatenate51/34
  t/6563 -> concatenate51/35
  t/6564 -> concatenate51/36
  t/6565 -> concatenate51/37
  t/6566 -> concatenate51/38
  t/6567 -> concatenate51/39
  t/6568 -> concatenate51/40
  t/6569 -> concatenate51/41
  t/6570 -> concatenate51/42
  t/6571 -> concatenate51/43
  t/6572 -> concatenate51/44
  t/6573 -> concatenate51/45
  t/6574 -> concatenate51/46
  t/6575 -> concatenate51/47
  t/6576 -> concatenate51/48
  t/6577 -> concatenate51/49
  t/6578 -> concatenate51/50
  t/6579 -> concatenate51/51
  t/6580 -> concatenate51/52
  t/6581 -> concatenate51/53
  t/6582 -> concatenate51/54
  t/6583 -> concatenate51/55
  t/6584 -> concatenate51/56
  t/6585 -> concatenate51/57
  t/6586 -> concatenate51/58
  t/6587 -> concatenate51/59
  t/6588 -> concatenate51/60
  t/6589 -> concatenate51/61
  t/6590 -> concatenate51/62
  t/6591 -> concatenate51/63
  t/6592 -> concatenate51/64
  t/6593 -> concatenate51/65
  t/6594 -> concatenate51/66
  t/6595 -> concatenate51/67
  t/6596 -> concatenate51/68
  t/6597 -> concatenate51/69
  t/6598 -> concatenate51/70
  t/6599 -> concatenate51/71
  t/6600 -> concatenate51/72
  t/6601 -> concatenate51/73
  t/6602 -> concatenate51/74
  t/6603 -> concatenate51/75
  t/6604 -> concatenate51/76
  t/6605 -> concatenate51/77
  t/6606 -> concatenate51/78
  t/6607 -> concatenate51/79
  t/6608 -> concatenate51/80
  t/6609 -> concatenate51/81
  t/6610 -> concatenate51/82
  t/6611 -> concatenate51/83
  t/6612 -> concatenate51/84
  t/6613 -> concatenate51/85
  t/6614 -> concatenate51/86
  t/6615 -> concatenate51/87
  t/6616 -> concatenate51/88
  t/6617 -> concatenate51/89
  t/6618 -> concatenate51/90
  t/6619 -> concatenate51/91
  t/6620 -> concatenate51/92
  t/6621 -> concatenate51/93
  t/6622 -> concatenate51/94
  t/6623 -> concatenate51/95
  t/6624 -> concatenate51/96
  t/6625 -> concatenate51/97
  t/6626 -> concatenate51/98
  t/6627 -> concatenate51/99
  t/6628 -> concatenate51/100
  t/6629 -> concatenate51/101
  t/6630 -> concatenate51/102
  t/6631 -> concatenate51/103
  t/6632 -> concatenate51/104
  t/6633 -> concatenate51/105
  t/6634 -> concatenate51/106
  t/6635 -> concatenate51/107
  t/6636 -> concatenate51/108
  t/6637 -> concatenate51/109
  t/6638 -> concatenate51/110
  t/6639 -> concatenate51/111
  t/6640 -> concatenate51/112
  t/6641 -> concatenate51/113
  t/6642 -> concatenate51/114
  t/6643 -> concatenate51/115
  t/6644 -> concatenate51/116
  t/6645 -> concatenate51/117
  t/6646 -> concatenate51/118
  t/6647 -> concatenate51/119
  t/6648 -> concatenate51/120
  t/6649 -> concatenate51/121
  t/6650 -> concatenate51/122
  t/6651 -> concatenate51/123
  t/6652 -> concatenate51/124
  t/6653 -> concatenate51/125
  t/6654 -> concatenate51/126
  t/6655 -> concatenate51/127
  t/6656 -> concatenate51/128
  t/6657 -> concatenate52/1
  t/6658 -> concatenate52/2
  t/6659 -> concatenate52/3
  t/6660 -> concatenate52/4
  t/6661 -> concatenate52/5
  t/6662 -> concatenate52/6
  t/6663 -> concatenate52/7
  t/6664 -> concatenate52/8
  t/6665 -> concatenate52/9
  t/6666 -> concatenate52/10
  t/6667 -> concatenate52/11
  t/6668 -> concatenate52/12
  t/6669 -> concatenate52/13
  t/6670 -> concatenate52/14
  t/6671 -> concatenate52/15
  t/6672 -> concatenate52/16
  t/6673 -> concatenate52/17
  t/6674 -> concatenate52/18
  t/6675 -> concatenate52/19
  t/6676 -> concatenate52/20
  t/6677 -> concatenate52/21
  t/6678 -> concatenate52/22
  t/6679 -> concatenate52/23
  t/6680 -> concatenate52/24
  t/6681 -> concatenate52/25
  t/6682 -> concatenate52/26
  t/6683 -> concatenate52/27
  t/6684 -> concatenate52/28
  t/6685 -> concatenate52/29
  t/6686 -> concatenate52/30
  t/6687 -> concatenate52/31
  t/6688 -> concatenate52/32
  t/6689 -> concatenate52/33
  t/6690 -> concatenate52/34
  t/6691 -> concatenate52/35
  t/6692 -> concatenate52/36
  t/6693 -> concatenate52/37
  t/6694 -> concatenate52/38
  t/6695 -> concatenate52/39
  t/6696 -> concatenate52/40
  t/6697 -> concatenate52/41
  t/6698 -> concatenate52/42
  t/6699 -> concatenate52/43
  t/6700 -> concatenate52/44
  t/6701 -> concatenate52/45
  t/6702 -> concatenate52/46
  t/6703 -> concatenate52/47
  t/6704 -> concatenate52/48
  t/6705 -> concatenate52/49
  t/6706 -> concatenate52/50
  t/6707 -> concatenate52/51
  t/6708 -> concatenate52/52
  t/6709 -> concatenate52/53
  t/6710 -> concatenate52/54
  t/6711 -> concatenate52/55
  t/6712 -> concatenate52/56
  t/6713 -> concatenate52/57
  t/6714 -> concatenate52/58
  t/6715 -> concatenate52/59
  t/6716 -> concatenate52/60
  t/6717 -> concatenate52/61
  t/6718 -> concatenate52/62
  t/6719 -> concatenate52/63
  t/6720 -> concatenate52/64
  t/6721 -> concatenate52/65
  t/6722 -> concatenate52/66
  t/6723 -> concatenate52/67
  t/6724 -> concatenate52/68
  t/6725 -> concatenate52/69
  t/6726 -> concatenate52/70
  t/6727 -> concatenate52/71
  t/6728 -> concatenate52/72
  t/6729 -> concatenate52/73
  t/6730 -> concatenate52/74
  t/6731 -> concatenate52/75
  t/6732 -> concatenate52/76
  t/6733 -> concatenate52/77
  t/6734 -> concatenate52/78
  t/6735 -> concatenate52/79
  t/6736 -> concatenate52/80
  t/6737 -> concatenate52/81
  t/6738 -> concatenate52/82
  t/6739 -> concatenate52/83
  t/6740 -> concatenate52/84
  t/6741 -> concatenate52/85
  t/6742 -> concatenate52/86
  t/6743 -> concatenate52/87
  t/6744 -> concatenate52/88
  t/6745 -> concatenate52/89
  t/6746 -> concatenate52/90
  t/6747 -> concatenate52/91
  t/6748 -> concatenate52/92
  t/6749 -> concatenate52/93
  t/6750 -> concatenate52/94
  t/6751 -> concatenate52/95
  t/6752 -> concatenate52/96
  t/6753 -> concatenate52/97
  t/6754 -> concatenate52/98
  t/6755 -> concatenate52/99
  t/6756 -> concatenate52/100
  t/6757 -> concatenate52/101
  t/6758 -> concatenate52/102
  t/6759 -> concatenate52/103
  t/6760 -> concatenate52/104
  t/6761 -> concatenate52/105
  t/6762 -> concatenate52/106
  t/6763 -> concatenate52/107
  t/6764 -> concatenate52/108
  t/6765 -> concatenate52/109
  t/6766 -> concatenate52/110
  t/6767 -> concatenate52/111
  t/6768 -> concatenate52/112
  t/6769 -> concatenate52/113
  t/6770 -> concatenate52/114
  t/6771 -> concatenate52/115
  t/6772 -> concatenate52/116
  t/6773 -> concatenate52/117
  t/6774 -> concatenate52/118
  t/6775 -> concatenate52/119
  t/6776 -> concatenate52/120
  t/6777 -> concatenate52/121
  t/6778 -> concatenate52/122
  t/6779 -> concatenate52/123
  t/6780 -> concatenate52/124
  t/6781 -> concatenate52/125
  t/6782 -> concatenate52/126
  t/6783 -> concatenate52/127
  t/6784 -> concatenate52/128
  t/6785 -> concatenate53/1
  t/6786 -> concatenate53/2
  t/6787 -> concatenate53/3
  t/6788 -> concatenate53/4
  t/6789 -> concatenate53/5
  t/6790 -> concatenate53/6
  t/6791 -> concatenate53/7
  t/6792 -> concatenate53/8
  t/6793 -> concatenate53/9
  t/6794 -> concatenate53/10
  t/6795 -> concatenate53/11
  t/6796 -> concatenate53/12
  t/6797 -> concatenate53/13
  t/6798 -> concatenate53/14
  t/6799 -> concatenate53/15
  t/6800 -> concatenate53/16
  t/6801 -> concatenate53/17
  t/6802 -> concatenate53/18
  t/6803 -> concatenate53/19
  t/6804 -> concatenate53/20
  t/6805 -> concatenate53/21
  t/6806 -> concatenate53/22
  t/6807 -> concatenate53/23
  t/6808 -> concatenate53/24
  t/6809 -> concatenate53/25
  t/6810 -> concatenate53/26
  t/6811 -> concatenate53/27
  t/6812 -> concatenate53/28
  t/6813 -> concatenate53/29
  t/6814 -> concatenate53/30
  t/6815 -> concatenate53/31
  t/6816 -> concatenate53/32
  t/6817 -> concatenate53/33
  t/6818 -> concatenate53/34
  t/6819 -> concatenate53/35
  t/6820 -> concatenate53/36
  t/6821 -> concatenate53/37
  t/6822 -> concatenate53/38
  t/6823 -> concatenate53/39
  t/6824 -> concatenate53/40
  t/6825 -> concatenate53/41
  t/6826 -> concatenate53/42
  t/6827 -> concatenate53/43
  t/6828 -> concatenate53/44
  t/6829 -> concatenate53/45
  t/6830 -> concatenate53/46
  t/6831 -> concatenate53/47
  t/6832 -> concatenate53/48
  t/6833 -> concatenate53/49
  t/6834 -> concatenate53/50
  t/6835 -> concatenate53/51
  t/6836 -> concatenate53/52
  t/6837 -> concatenate53/53
  t/6838 -> concatenate53/54
  t/6839 -> concatenate53/55
  t/6840 -> concatenate53/56
  t/6841 -> concatenate53/57
  t/6842 -> concatenate53/58
  t/6843 -> concatenate53/59
  t/6844 -> concatenate53/60
  t/6845 -> concatenate53/61
  t/6846 -> concatenate53/62
  t/6847 -> concatenate53/63
  t/6848 -> concatenate53/64
  t/6849 -> concatenate53/65
  t/6850 -> concatenate53/66
  t/6851 -> concatenate53/67
  t/6852 -> concatenate53/68
  t/6853 -> concatenate53/69
  t/6854 -> concatenate53/70
  t/6855 -> concatenate53/71
  t/6856 -> concatenate53/72
  t/6857 -> concatenate53/73
  t/6858 -> concatenate53/74
  t/6859 -> concatenate53/75
  t/6860 -> concatenate53/76
  t/6861 -> concatenate53/77
  t/6862 -> concatenate53/78
  t/6863 -> concatenate53/79
  t/6864 -> concatenate53/80
  t/6865 -> concatenate53/81
  t/6866 -> concatenate53/82
  t/6867 -> concatenate53/83
  t/6868 -> concatenate53/84
  t/6869 -> concatenate53/85
  t/6870 -> concatenate53/86
  t/6871 -> concatenate53/87
  t/6872 -> concatenate53/88
  t/6873 -> concatenate53/89
  t/6874 -> concatenate53/90
  t/6875 -> concatenate53/91
  t/6876 -> concatenate53/92
  t/6877 -> concatenate53/93
  t/6878 -> concatenate53/94
  t/6879 -> concatenate53/95
  t/6880 -> concatenate53/96
  t/6881 -> concatenate53/97
  t/6882 -> concatenate53/98
  t/6883 -> concatenate53/99
  t/6884 -> concatenate53/100
  t/6885 -> concatenate53/101
  t/6886 -> concatenate53/102
  t/6887 -> concatenate53/103
  t/6888 -> concatenate53/104
  t/6889 -> concatenate53/105
  t/6890 -> concatenate53/106
  t/6891 -> concatenate53/107
  t/6892 -> concatenate53/108
  t/6893 -> concatenate53/109
  t/6894 -> concatenate53/110
  t/6895 -> concatenate53/111
  t/6896 -> concatenate53/112
  t/6897 -> concatenate53/113
  t/6898 -> concatenate53/114
  t/6899 -> concatenate53/115
  t/6900 -> concatenate53/116
  t/6901 -> concatenate53/117
  t/6902 -> concatenate53/118
  t/6903 -> concatenate53/119
  t/6904 -> concatenate53/120
  t/6905 -> concatenate53/121
  t/6906 -> concatenate53/122
  t/6907 -> concatenate53/123
  t/6908 -> concatenate53/124
  t/6909 -> concatenate53/125
  t/6910 -> concatenate53/126
  t/6911 -> concatenate53/127
  t/6912 -> concatenate53/128
  t/6913 -> concatenate54/1
  t/6914 -> concatenate54/2
  t/6915 -> concatenate54/3
  t/6916 -> concatenate54/4
  t/6917 -> concatenate54/5
  t/6918 -> concatenate54/6
  t/6919 -> concatenate54/7
  t/6920 -> concatenate54/8
  t/6921 -> concatenate54/9
  t/6922 -> concatenate54/10
  t/6923 -> concatenate54/11
  t/6924 -> concatenate54/12
  t/6925 -> concatenate54/13
  t/6926 -> concatenate54/14
  t/6927 -> concatenate54/15
  t/6928 -> concatenate54/16
  t/6929 -> concatenate54/17
  t/6930 -> concatenate54/18
  t/6931 -> concatenate54/19
  t/6932 -> concatenate54/20
  t/6933 -> concatenate54/21
  t/6934 -> concatenate54/22
  t/6935 -> concatenate54/23
  t/6936 -> concatenate54/24
  t/6937 -> concatenate54/25
  t/6938 -> concatenate54/26
  t/6939 -> concatenate54/27
  t/6940 -> concatenate54/28
  t/6941 -> concatenate54/29
  t/6942 -> concatenate54/30
  t/6943 -> concatenate54/31
  t/6944 -> concatenate54/32
  t/6945 -> concatenate54/33
  t/6946 -> concatenate54/34
  t/6947 -> concatenate54/35
  t/6948 -> concatenate54/36
  t/6949 -> concatenate54/37
  t/6950 -> concatenate54/38
  t/6951 -> concatenate54/39
  t/6952 -> concatenate54/40
  t/6953 -> concatenate54/41
  t/6954 -> concatenate54/42
  t/6955 -> concatenate54/43
  t/6956 -> concatenate54/44
  t/6957 -> concatenate54/45
  t/6958 -> concatenate54/46
  t/6959 -> concatenate54/47
  t/6960 -> concatenate54/48
  t/6961 -> concatenate54/49
  t/6962 -> concatenate54/50
  t/6963 -> concatenate54/51
  t/6964 -> concatenate54/52
  t/6965 -> concatenate54/53
  t/6966 -> concatenate54/54
  t/6967 -> concatenate54/55
  t/6968 -> concatenate54/56
  t/6969 -> concatenate54/57
  t/6970 -> concatenate54/58
  t/6971 -> concatenate54/59
  t/6972 -> concatenate54/60
  t/6973 -> concatenate54/61
  t/6974 -> concatenate54/62
  t/6975 -> concatenate54/63
  t/6976 -> concatenate54/64
  t/6977 -> concatenate54/65
  t/6978 -> concatenate54/66
  t/6979 -> concatenate54/67
  t/6980 -> concatenate54/68
  t/6981 -> concatenate54/69
  t/6982 -> concatenate54/70
  t/6983 -> concatenate54/71
  t/6984 -> concatenate54/72
  t/6985 -> concatenate54/73
  t/6986 -> concatenate54/74
  t/6987 -> concatenate54/75
  t/6988 -> concatenate54/76
  t/6989 -> concatenate54/77
  t/6990 -> concatenate54/78
  t/6991 -> concatenate54/79
  t/6992 -> concatenate54/80
  t/6993 -> concatenate54/81
  t/6994 -> concatenate54/82
  t/6995 -> concatenate54/83
  t/6996 -> concatenate54/84
  t/6997 -> concatenate54/85
  t/6998 -> concatenate54/86
  t/6999 -> concatenate54/87
  t/7000 -> concatenate54/88
  t/7001 -> concatenate54/89
  t/7002 -> concatenate54/90
  t/7003 -> concatenate54/91
  t/7004 -> concatenate54/92
  t/7005 -> concatenate54/93
  t/7006 -> concatenate54/94
  t/7007 -> concatenate54/95
  t/7008 -> concatenate54/96
  t/7009 -> concatenate54/97
  t/7010 -> concatenate54/98
  t/7011 -> concatenate54/99
  t/7012 -> concatenate54/100
  t/7013 -> concatenate54/101
  t/7014 -> concatenate54/102
  t/7015 -> concatenate54/103
  t/7016 -> concatenate54/104
  t/7017 -> concatenate54/105
  t/7018 -> concatenate54/106
  t/7019 -> concatenate54/107
  t/7020 -> concatenate54/108
  t/7021 -> concatenate54/109
  t/7022 -> concatenate54/110
  t/7023 -> concatenate54/111
  t/7024 -> concatenate54/112
  t/7025 -> concatenate54/113
  t/7026 -> concatenate54/114
  t/7027 -> concatenate54/115
  t/7028 -> concatenate54/116
  t/7029 -> concatenate54/117
  t/7030 -> concatenate54/118
  t/7031 -> concatenate54/119
  t/7032 -> concatenate54/120
  t/7033 -> concatenate54/121
  t/7034 -> concatenate54/122
  t/7035 -> concatenate54/123
  t/7036 -> concatenate54/124
  t/7037 -> concatenate54/125
  t/7038 -> concatenate54/126
  t/7039 -> concatenate54/127
  t/7040 -> concatenate54/128
  t/7041 -> concatenate55/1
  t/7042 -> concatenate55/2
  t/7043 -> concatenate55/3
  t/7044 -> concatenate55/4
  t/7045 -> concatenate55/5
  t/7046 -> concatenate55/6
  t/7047 -> concatenate55/7
  t/7048 -> concatenate55/8
  t/7049 -> concatenate55/9
  t/7050 -> concatenate55/10
  t/7051 -> concatenate55/11
  t/7052 -> concatenate55/12
  t/7053 -> concatenate55/13
  t/7054 -> concatenate55/14
  t/7055 -> concatenate55/15
  t/7056 -> concatenate55/16
  t/7057 -> concatenate55/17
  t/7058 -> concatenate55/18
  t/7059 -> concatenate55/19
  t/7060 -> concatenate55/20
  t/7061 -> concatenate55/21
  t/7062 -> concatenate55/22
  t/7063 -> concatenate55/23
  t/7064 -> concatenate55/24
  t/7065 -> concatenate55/25
  t/7066 -> concatenate55/26
  t/7067 -> concatenate55/27
  t/7068 -> concatenate55/28
  t/7069 -> concatenate55/29
  t/7070 -> concatenate55/30
  t/7071 -> concatenate55/31
  t/7072 -> concatenate55/32
  t/7073 -> concatenate55/33
  t/7074 -> concatenate55/34
  t/7075 -> concatenate55/35
  t/7076 -> concatenate55/36
  t/7077 -> concatenate55/37
  t/7078 -> concatenate55/38
  t/7079 -> concatenate55/39
  t/7080 -> concatenate55/40
  t/7081 -> concatenate55/41
  t/7082 -> concatenate55/42
  t/7083 -> concatenate55/43
  t/7084 -> concatenate55/44
  t/7085 -> concatenate55/45
  t/7086 -> concatenate55/46
  t/7087 -> concatenate55/47
  t/7088 -> concatenate55/48
  t/7089 -> concatenate55/49
  t/7090 -> concatenate55/50
  t/7091 -> concatenate55/51
  t/7092 -> concatenate55/52
  t/7093 -> concatenate55/53
  t/7094 -> concatenate55/54
  t/7095 -> concatenate55/55
  t/7096 -> concatenate55/56
  t/7097 -> concatenate55/57
  t/7098 -> concatenate55/58
  t/7099 -> concatenate55/59
  t/7100 -> concatenate55/60
  t/7101 -> concatenate55/61
  t/7102 -> concatenate55/62
  t/7103 -> concatenate55/63
  t/7104 -> concatenate55/64
  t/7105 -> concatenate55/65
  t/7106 -> concatenate55/66
  t/7107 -> concatenate55/67
  t/7108 -> concatenate55/68
  t/7109 -> concatenate55/69
  t/7110 -> concatenate55/70
  t/7111 -> concatenate55/71
  t/7112 -> concatenate55/72
  t/7113 -> concatenate55/73
  t/7114 -> concatenate55/74
  t/7115 -> concatenate55/75
  t/7116 -> concatenate55/76
  t/7117 -> concatenate55/77
  t/7118 -> concatenate55/78
  t/7119 -> concatenate55/79
  t/7120 -> concatenate55/80
  t/7121 -> concatenate55/81
  t/7122 -> concatenate55/82
  t/7123 -> concatenate55/83
  t/7124 -> concatenate55/84
  t/7125 -> concatenate55/85
  t/7126 -> concatenate55/86
  t/7127 -> concatenate55/87
  t/7128 -> concatenate55/88
  t/7129 -> concatenate55/89
  t/7130 -> concatenate55/90
  t/7131 -> concatenate55/91
  t/7132 -> concatenate55/92
  t/7133 -> concatenate55/93
  t/7134 -> concatenate55/94
  t/7135 -> concatenate55/95
  t/7136 -> concatenate55/96
  t/7137 -> concatenate55/97
  t/7138 -> concatenate55/98
  t/7139 -> concatenate55/99
  t/7140 -> concatenate55/100
  t/7141 -> concatenate55/101
  t/7142 -> concatenate55/102
  t/7143 -> concatenate55/103
  t/7144 -> concatenate55/104
  t/7145 -> concatenate55/105
  t/7146 -> concatenate55/106
  t/7147 -> concatenate55/107
  t/7148 -> concatenate55/108
  t/7149 -> concatenate55/109
  t/7150 -> concatenate55/110
  t/7151 -> concatenate55/111
  t/7152 -> concatenate55/112
  t/7153 -> concatenate55/113
  t/7154 -> concatenate55/114
  t/7155 -> concatenate55/115
  t/7156 -> concatenate55/116
  t/7157 -> concatenate55/117
  t/7158 -> concatenate55/118
  t/7159 -> concatenate55/119
  t/7160 -> concatenate55/120
  t/7161 -> concatenate55/121
  t/7162 -> concatenate55/122
  t/7163 -> concatenate55/123
  t/7164 -> concatenate55/124
  t/7165 -> concatenate55/125
  t/7166 -> concatenate55/126
  t/7167 -> concatenate55/127
  t/7168 -> concatenate55/128
  t/7169 -> concatenate56/1
  t/7170 -> concatenate56/2
  t/7171 -> concatenate56/3
  t/7172 -> concatenate56/4
  t/7173 -> concatenate56/5
  t/7174 -> concatenate56/6
  t/7175 -> concatenate56/7
  t/7176 -> concatenate56/8
  t/7177 -> concatenate56/9
  t/7178 -> concatenate56/10
  t/7179 -> concatenate56/11
  t/7180 -> concatenate56/12
  t/7181 -> concatenate56/13
  t/7182 -> concatenate56/14
  t/7183 -> concatenate56/15
  t/7184 -> concatenate56/16
  t/7185 -> concatenate56/17
  t/7186 -> concatenate56/18
  t/7187 -> concatenate56/19
  t/7188 -> concatenate56/20
  t/7189 -> concatenate56/21
  t/7190 -> concatenate56/22
  t/7191 -> concatenate56/23
  t/7192 -> concatenate56/24
  t/7193 -> concatenate56/25
  t/7194 -> concatenate56/26
  t/7195 -> concatenate56/27
  t/7196 -> concatenate56/28
  t/7197 -> concatenate56/29
  t/7198 -> concatenate56/30
  t/7199 -> concatenate56/31
  t/7200 -> concatenate56/32
  t/7201 -> concatenate56/33
  t/7202 -> concatenate56/34
  t/7203 -> concatenate56/35
  t/7204 -> concatenate56/36
  t/7205 -> concatenate56/37
  t/7206 -> concatenate56/38
  t/7207 -> concatenate56/39
  t/7208 -> concatenate56/40
  t/7209 -> concatenate56/41
  t/7210 -> concatenate56/42
  t/7211 -> concatenate56/43
  t/7212 -> concatenate56/44
  t/7213 -> concatenate56/45
  t/7214 -> concatenate56/46
  t/7215 -> concatenate56/47
  t/7216 -> concatenate56/48
  t/7217 -> concatenate56/49
  t/7218 -> concatenate56/50
  t/7219 -> concatenate56/51
  t/7220 -> concatenate56/52
  t/7221 -> concatenate56/53
  t/7222 -> concatenate56/54
  t/7223 -> concatenate56/55
  t/7224 -> concatenate56/56
  t/7225 -> concatenate56/57
  t/7226 -> concatenate56/58
  t/7227 -> concatenate56/59
  t/7228 -> concatenate56/60
  t/7229 -> concatenate56/61
  t/7230 -> concatenate56/62
  t/7231 -> concatenate56/63
  t/7232 -> concatenate56/64
  t/7233 -> concatenate56/65
  t/7234 -> concatenate56/66
  t/7235 -> concatenate56/67
  t/7236 -> concatenate56/68
  t/7237 -> concatenate56/69
  t/7238 -> concatenate56/70
  t/7239 -> concatenate56/71
  t/7240 -> concatenate56/72
  t/7241 -> concatenate56/73
  t/7242 -> concatenate56/74
  t/7243 -> concatenate56/75
  t/7244 -> concatenate56/76
  t/7245 -> concatenate56/77
  t/7246 -> concatenate56/78
  t/7247 -> concatenate56/79
  t/7248 -> concatenate56/80
  t/7249 -> concatenate56/81
  t/7250 -> concatenate56/82
  t/7251 -> concatenate56/83
  t/7252 -> concatenate56/84
  t/7253 -> concatenate56/85
  t/7254 -> concatenate56/86
  t/7255 -> concatenate56/87
  t/7256 -> concatenate56/88
  t/7257 -> concatenate56/89
  t/7258 -> concatenate56/90
  t/7259 -> concatenate56/91
  t/7260 -> concatenate56/92
  t/7261 -> concatenate56/93
  t/7262 -> concatenate56/94
  t/7263 -> concatenate56/95
  t/7264 -> concatenate56/96
  t/7265 -> concatenate56/97
  t/7266 -> concatenate56/98
  t/7267 -> concatenate56/99
  t/7268 -> concatenate56/100
  t/7269 -> concatenate56/101
  t/7270 -> concatenate56/102
  t/7271 -> concatenate56/103
  t/7272 -> concatenate56/104
  t/7273 -> concatenate56/105
  t/7274 -> concatenate56/106
  t/7275 -> concatenate56/107
  t/7276 -> concatenate56/108
  t/7277 -> concatenate56/109
  t/7278 -> concatenate56/110
  t/7279 -> concatenate56/111
  t/7280 -> concatenate56/112
  t/7281 -> concatenate56/113
  t/7282 -> concatenate56/114
  t/7283 -> concatenate56/115
  t/7284 -> concatenate56/116
  t/7285 -> concatenate56/117
  t/7286 -> concatenate56/118
  t/7287 -> concatenate56/119
  t/7288 -> concatenate56/120
  t/7289 -> concatenate56/121
  t/7290 -> concatenate56/122
  t/7291 -> concatenate56/123
  t/7292 -> concatenate56/124
  t/7293 -> concatenate56/125
  t/7294 -> concatenate56/126
  t/7295 -> concatenate56/127
  t/7296 -> concatenate56/128
  t/7297 -> concatenate57/1
  t/7298 -> concatenate57/2
  t/7299 -> concatenate57/3
  t/7300 -> concatenate57/4
  t/7301 -> concatenate57/5
  t/7302 -> concatenate57/6
  t/7303 -> concatenate57/7
  t/7304 -> concatenate57/8
  t/7305 -> concatenate57/9
  t/7306 -> concatenate57/10
  t/7307 -> concatenate57/11
  t/7308 -> concatenate57/12
  t/7309 -> concatenate57/13
  t/7310 -> concatenate57/14
  t/7311 -> concatenate57/15
  t/7312 -> concatenate57/16
  t/7313 -> concatenate57/17
  t/7314 -> concatenate57/18
  t/7315 -> concatenate57/19
  t/7316 -> concatenate57/20
  t/7317 -> concatenate57/21
  t/7318 -> concatenate57/22
  t/7319 -> concatenate57/23
  t/7320 -> concatenate57/24
  t/7321 -> concatenate57/25
  t/7322 -> concatenate57/26
  t/7323 -> concatenate57/27
  t/7324 -> concatenate57/28
  t/7325 -> concatenate57/29
  t/7326 -> concatenate57/30
  t/7327 -> concatenate57/31
  t/7328 -> concatenate57/32
  t/7329 -> concatenate57/33
  t/7330 -> concatenate57/34
  t/7331 -> concatenate57/35
  t/7332 -> concatenate57/36
  t/7333 -> concatenate57/37
  t/7334 -> concatenate57/38
  t/7335 -> concatenate57/39
  t/7336 -> concatenate57/40
  t/7337 -> concatenate57/41
  t/7338 -> concatenate57/42
  t/7339 -> concatenate57/43
  t/7340 -> concatenate57/44
  t/7341 -> concatenate57/45
  t/7342 -> concatenate57/46
  t/7343 -> concatenate57/47
  t/7344 -> concatenate57/48
  t/7345 -> concatenate57/49
  t/7346 -> concatenate57/50
  t/7347 -> concatenate57/51
  t/7348 -> concatenate57/52
  t/7349 -> concatenate57/53
  t/7350 -> concatenate57/54
  t/7351 -> concatenate57/55
  t/7352 -> concatenate57/56
  t/7353 -> concatenate57/57
  t/7354 -> concatenate57/58
  t/7355 -> concatenate57/59
  t/7356 -> concatenate57/60
  t/7357 -> concatenate57/61
  t/7358 -> concatenate57/62
  t/7359 -> concatenate57/63
  t/7360 -> concatenate57/64
  t/7361 -> concatenate57/65
  t/7362 -> concatenate57/66
  t/7363 -> concatenate57/67
  t/7364 -> concatenate57/68
  t/7365 -> concatenate57/69
  t/7366 -> concatenate57/70
  t/7367 -> concatenate57/71
  t/7368 -> concatenate57/72
  t/7369 -> concatenate57/73
  t/7370 -> concatenate57/74
  t/7371 -> concatenate57/75
  t/7372 -> concatenate57/76
  t/7373 -> concatenate57/77
  t/7374 -> concatenate57/78
  t/7375 -> concatenate57/79
  t/7376 -> concatenate57/80
  t/7377 -> concatenate57/81
  t/7378 -> concatenate57/82
  t/7379 -> concatenate57/83
  t/7380 -> concatenate57/84
  t/7381 -> concatenate57/85
  t/7382 -> concatenate57/86
  t/7383 -> concatenate57/87
  t/7384 -> concatenate57/88
  t/7385 -> concatenate57/89
  t/7386 -> concatenate57/90
  t/7387 -> concatenate57/91
  t/7388 -> concatenate57/92
  t/7389 -> concatenate57/93
  t/7390 -> concatenate57/94
  t/7391 -> concatenate57/95
  t/7392 -> concatenate57/96
  t/7393 -> concatenate57/97
  t/7394 -> concatenate57/98
  t/7395 -> concatenate57/99
  t/7396 -> concatenate57/100
  t/7397 -> concatenate57/101
  t/7398 -> concatenate57/102
  t/7399 -> concatenate57/103
  t/7400 -> concatenate57/104
  t/7401 -> concatenate57/105
  t/7402 -> concatenate57/106
  t/7403 -> concatenate57/107
  t/7404 -> concatenate57/108
  t/7405 -> concatenate57/109
  t/7406 -> concatenate57/110
  t/7407 -> concatenate57/111
  t/7408 -> concatenate57/112
  t/7409 -> concatenate57/113
  t/7410 -> concatenate57/114
  t/7411 -> concatenate57/115
  t/7412 -> concatenate57/116
  t/7413 -> concatenate57/117
  t/7414 -> concatenate57/118
  t/7415 -> concatenate57/119
  t/7416 -> concatenate57/120
  t/7417 -> concatenate57/121
  t/7418 -> concatenate57/122
  t/7419 -> concatenate57/123
  t/7420 -> concatenate57/124
  t/7421 -> concatenate57/125
  t/7422 -> concatenate57/126
  t/7423 -> concatenate57/127
  t/7424 -> concatenate57/128
  t/7425 -> concatenate58/1
  t/7426 -> concatenate58/2
  t/7427 -> concatenate58/3
  t/7428 -> concatenate58/4
  t/7429 -> concatenate58/5
  t/7430 -> concatenate58/6
  t/7431 -> concatenate58/7
  t/7432 -> concatenate58/8
  t/7433 -> concatenate58/9
  t/7434 -> concatenate58/10
  t/7435 -> concatenate58/11
  t/7436 -> concatenate58/12
  t/7437 -> concatenate58/13
  t/7438 -> concatenate58/14
  t/7439 -> concatenate58/15
  t/7440 -> concatenate58/16
  t/7441 -> concatenate58/17
  t/7442 -> concatenate58/18
  t/7443 -> concatenate58/19
  t/7444 -> concatenate58/20
  t/7445 -> concatenate58/21
  t/7446 -> concatenate58/22
  t/7447 -> concatenate58/23
  t/7448 -> concatenate58/24
  t/7449 -> concatenate58/25
  t/7450 -> concatenate58/26
  t/7451 -> concatenate58/27
  t/7452 -> concatenate58/28
  t/7453 -> concatenate58/29
  t/7454 -> concatenate58/30
  t/7455 -> concatenate58/31
  t/7456 -> concatenate58/32
  t/7457 -> concatenate58/33
  t/7458 -> concatenate58/34
  t/7459 -> concatenate58/35
  t/7460 -> concatenate58/36
  t/7461 -> concatenate58/37
  t/7462 -> concatenate58/38
  t/7463 -> concatenate58/39
  t/7464 -> concatenate58/40
  t/7465 -> concatenate58/41
  t/7466 -> concatenate58/42
  t/7467 -> concatenate58/43
  t/7468 -> concatenate58/44
  t/7469 -> concatenate58/45
  t/7470 -> concatenate58/46
  t/7471 -> concatenate58/47
  t/7472 -> concatenate58/48
  t/7473 -> concatenate58/49
  t/7474 -> concatenate58/50
  t/7475 -> concatenate58/51
  t/7476 -> concatenate58/52
  t/7477 -> concatenate58/53
  t/7478 -> concatenate58/54
  t/7479 -> concatenate58/55
  t/7480 -> concatenate58/56
  t/7481 -> concatenate58/57
  t/7482 -> concatenate58/58
  t/7483 -> concatenate58/59
  t/7484 -> concatenate58/60
  t/7485 -> concatenate58/61
  t/7486 -> concatenate58/62
  t/7487 -> concatenate58/63
  t/7488 -> concatenate58/64
  t/7489 -> concatenate58/65
  t/7490 -> concatenate58/66
  t/7491 -> concatenate58/67
  t/7492 -> concatenate58/68
  t/7493 -> concatenate58/69
  t/7494 -> concatenate58/70
  t/7495 -> concatenate58/71
  t/7496 -> concatenate58/72
  t/7497 -> concatenate58/73
  t/7498 -> concatenate58/74
  t/7499 -> concatenate58/75
  t/7500 -> concatenate58/76
  t/7501 -> concatenate58/77
  t/7502 -> concatenate58/78
  t/7503 -> concatenate58/79
  t/7504 -> concatenate58/80
  t/7505 -> concatenate58/81
  t/7506 -> concatenate58/82
  t/7507 -> concatenate58/83
  t/7508 -> concatenate58/84
  t/7509 -> concatenate58/85
  t/7510 -> concatenate58/86
  t/7511 -> concatenate58/87
  t/7512 -> concatenate58/88
  t/7513 -> concatenate58/89
  t/7514 -> concatenate58/90
  t/7515 -> concatenate58/91
  t/7516 -> concatenate58/92
  t/7517 -> concatenate58/93
  t/7518 -> concatenate58/94
  t/7519 -> concatenate58/95
  t/7520 -> concatenate58/96
  t/7521 -> concatenate58/97
  t/7522 -> concatenate58/98
  t/7523 -> concatenate58/99
  t/7524 -> concatenate58/100
  t/7525 -> concatenate58/101
  t/7526 -> concatenate58/102
  t/7527 -> concatenate58/103
  t/7528 -> concatenate58/104
  t/7529 -> concatenate58/105
  t/7530 -> concatenate58/106
  t/7531 -> concatenate58/107
  t/7532 -> concatenate58/108
  t/7533 -> concatenate58/109
  t/7534 -> concatenate58/110
  t/7535 -> concatenate58/111
  t/7536 -> concatenate58/112
  t/7537 -> concatenate58/113
  t/7538 -> concatenate58/114
  t/7539 -> concatenate58/115
  t/7540 -> concatenate58/116
  t/7541 -> concatenate58/117
  t/7542 -> concatenate58/118
  t/7543 -> concatenate58/119
  t/7544 -> concatenate58/120
  t/7545 -> concatenate58/121
  t/7546 -> concatenate58/122
  t/7547 -> concatenate58/123
  t/7548 -> concatenate58/124
  t/7549 -> concatenate58/125
  t/7550 -> concatenate58/126
  t/7551 -> concatenate58/127
  t/7552 -> concatenate58/128
  t/7553 -> concatenate59/1
  t/7554 -> concatenate59/2
  t/7555 -> concatenate59/3
  t/7556 -> concatenate59/4
  t/7557 -> concatenate59/5
  t/7558 -> concatenate59/6
  t/7559 -> concatenate59/7
  t/7560 -> concatenate59/8
  t/7561 -> concatenate59/9
  t/7562 -> concatenate59/10
  t/7563 -> concatenate59/11
  t/7564 -> concatenate59/12
  t/7565 -> concatenate59/13
  t/7566 -> concatenate59/14
  t/7567 -> concatenate59/15
  t/7568 -> concatenate59/16
  t/7569 -> concatenate59/17
  t/7570 -> concatenate59/18
  t/7571 -> concatenate59/19
  t/7572 -> concatenate59/20
  t/7573 -> concatenate59/21
  t/7574 -> concatenate59/22
  t/7575 -> concatenate59/23
  t/7576 -> concatenate59/24
  t/7577 -> concatenate59/25
  t/7578 -> concatenate59/26
  t/7579 -> concatenate59/27
  t/7580 -> concatenate59/28
  t/7581 -> concatenate59/29
  t/7582 -> concatenate59/30
  t/7583 -> concatenate59/31
  t/7584 -> concatenate59/32
  t/7585 -> concatenate59/33
  t/7586 -> concatenate59/34
  t/7587 -> concatenate59/35
  t/7588 -> concatenate59/36
  t/7589 -> concatenate59/37
  t/7590 -> concatenate59/38
  t/7591 -> concatenate59/39
  t/7592 -> concatenate59/40
  t/7593 -> concatenate59/41
  t/7594 -> concatenate59/42
  t/7595 -> concatenate59/43
  t/7596 -> concatenate59/44
  t/7597 -> concatenate59/45
  t/7598 -> concatenate59/46
  t/7599 -> concatenate59/47
  t/7600 -> concatenate59/48
  t/7601 -> concatenate59/49
  t/7602 -> concatenate59/50
  t/7603 -> concatenate59/51
  t/7604 -> concatenate59/52
  t/7605 -> concatenate59/53
  t/7606 -> concatenate59/54
  t/7607 -> concatenate59/55
  t/7608 -> concatenate59/56
  t/7609 -> concatenate59/57
  t/7610 -> concatenate59/58
  t/7611 -> concatenate59/59
  t/7612 -> concatenate59/60
  t/7613 -> concatenate59/61
  t/7614 -> concatenate59/62
  t/7615 -> concatenate59/63
  t/7616 -> concatenate59/64
  t/7617 -> concatenate59/65
  t/7618 -> concatenate59/66
  t/7619 -> concatenate59/67
  t/7620 -> concatenate59/68
  t/7621 -> concatenate59/69
  t/7622 -> concatenate59/70
  t/7623 -> concatenate59/71
  t/7624 -> concatenate59/72
  t/7625 -> concatenate59/73
  t/7626 -> concatenate59/74
  t/7627 -> concatenate59/75
  t/7628 -> concatenate59/76
  t/7629 -> concatenate59/77
  t/7630 -> concatenate59/78
  t/7631 -> concatenate59/79
  t/7632 -> concatenate59/80
  t/7633 -> concatenate59/81
  t/7634 -> concatenate59/82
  t/7635 -> concatenate59/83
  t/7636 -> concatenate59/84
  t/7637 -> concatenate59/85
  t/7638 -> concatenate59/86
  t/7639 -> concatenate59/87
  t/7640 -> concatenate59/88
  t/7641 -> concatenate59/89
  t/7642 -> concatenate59/90
  t/7643 -> concatenate59/91
  t/7644 -> concatenate59/92
  t/7645 -> concatenate59/93
  t/7646 -> concatenate59/94
  t/7647 -> concatenate59/95
  t/7648 -> concatenate59/96
  t/7649 -> concatenate59/97
  t/7650 -> concatenate59/98
  t/7651 -> concatenate59/99
  t/7652 -> concatenate59/100
  t/7653 -> concatenate59/101
  t/7654 -> concatenate59/102
  t/7655 -> concatenate59/103
  t/7656 -> concatenate59/104
  t/7657 -> concatenate59/105
  t/7658 -> concatenate59/106
  t/7659 -> concatenate59/107
  t/7660 -> concatenate59/108
  t/7661 -> concatenate59/109
  t/7662 -> concatenate59/110
  t/7663 -> concatenate59/111
  t/7664 -> concatenate59/112
  t/7665 -> concatenate59/113
  t/7666 -> concatenate59/114
  t/7667 -> concatenate59/115
  t/7668 -> concatenate59/116
  t/7669 -> concatenate59/117
  t/7670 -> concatenate59/118
  t/7671 -> concatenate59/119
  t/7672 -> concatenate59/120
  t/7673 -> concatenate59/121
  t/7674 -> concatenate59/122
  t/7675 -> concatenate59/123
  t/7676 -> concatenate59/124
  t/7677 -> concatenate59/125
  t/7678 -> concatenate59/126
  t/7679 -> concatenate59/127
  t/7680 -> concatenate59/128
  t/7681 -> concatenate60/1
  t/7682 -> concatenate60/2
  t/7683 -> concatenate60/3
  t/7684 -> concatenate60/4
  t/7685 -> concatenate60/5
  t/7686 -> concatenate60/6
  t/7687 -> concatenate60/7
  t/7688 -> concatenate60/8
  t/7689 -> concatenate60/9
  t/7690 -> concatenate60/10
  t/7691 -> concatenate60/11
  t/7692 -> concatenate60/12
  t/7693 -> concatenate60/13
  t/7694 -> concatenate60/14
  t/7695 -> concatenate60/15
  t/7696 -> concatenate60/16
  t/7697 -> concatenate60/17
  t/7698 -> concatenate60/18
  t/7699 -> concatenate60/19
  t/7700 -> concatenate60/20
  t/7701 -> concatenate60/21
  t/7702 -> concatenate60/22
  t/7703 -> concatenate60/23
  t/7704 -> concatenate60/24
  t/7705 -> concatenate60/25
  t/7706 -> concatenate60/26
  t/7707 -> concatenate60/27
  t/7708 -> concatenate60/28
  t/7709 -> concatenate60/29
  t/7710 -> concatenate60/30
  t/7711 -> concatenate60/31
  t/7712 -> concatenate60/32
  t/7713 -> concatenate60/33
  t/7714 -> concatenate60/34
  t/7715 -> concatenate60/35
  t/7716 -> concatenate60/36
  t/7717 -> concatenate60/37
  t/7718 -> concatenate60/38
  t/7719 -> concatenate60/39
  t/7720 -> concatenate60/40
  t/7721 -> concatenate60/41
  t/7722 -> concatenate60/42
  t/7723 -> concatenate60/43
  t/7724 -> concatenate60/44
  t/7725 -> concatenate60/45
  t/7726 -> concatenate60/46
  t/7727 -> concatenate60/47
  t/7728 -> concatenate60/48
  t/7729 -> concatenate60/49
  t/7730 -> concatenate60/50
  t/7731 -> concatenate60/51
  t/7732 -> concatenate60/52
  t/7733 -> concatenate60/53
  t/7734 -> concatenate60/54
  t/7735 -> concatenate60/55
  t/7736 -> concatenate60/56
  t/7737 -> concatenate60/57
  t/7738 -> concatenate60/58
  t/7739 -> concatenate60/59
  t/7740 -> concatenate60/60
  t/7741 -> concatenate60/61
  t/7742 -> concatenate60/62
  t/7743 -> concatenate60/63
  t/7744 -> concatenate60/64
  t/7745 -> concatenate60/65
  t/7746 -> concatenate60/66
  t/7747 -> concatenate60/67
  t/7748 -> concatenate60/68
  t/7749 -> concatenate60/69
  t/7750 -> concatenate60/70
  t/7751 -> concatenate60/71
  t/7752 -> concatenate60/72
  t/7753 -> concatenate60/73
  t/7754 -> concatenate60/74
  t/7755 -> concatenate60/75
  t/7756 -> concatenate60/76
  t/7757 -> concatenate60/77
  t/7758 -> concatenate60/78
  t/7759 -> concatenate60/79
  t/7760 -> concatenate60/80
  t/7761 -> concatenate60/81
  t/7762 -> concatenate60/82
  t/7763 -> concatenate60/83
  t/7764 -> concatenate60/84
  t/7765 -> concatenate60/85
  t/7766 -> concatenate60/86
  t/7767 -> concatenate60/87
  t/7768 -> concatenate60/88
  t/7769 -> concatenate60/89
  t/7770 -> concatenate60/90
  t/7771 -> concatenate60/91
  t/7772 -> concatenate60/92
  t/7773 -> concatenate60/93
  t/7774 -> concatenate60/94
  t/7775 -> concatenate60/95
  t/7776 -> concatenate60/96
  t/7777 -> concatenate60/97
  t/7778 -> concatenate60/98
  t/7779 -> concatenate60/99
  t/7780 -> concatenate60/100
  t/7781 -> concatenate60/101
  t/7782 -> concatenate60/102
  t/7783 -> concatenate60/103
  t/7784 -> concatenate60/104
  t/7785 -> concatenate60/105
  t/7786 -> concatenate60/106
  t/7787 -> concatenate60/107
  t/7788 -> concatenate60/108
  t/7789 -> concatenate60/109
  t/7790 -> concatenate60/110
  t/7791 -> concatenate60/111
  t/7792 -> concatenate60/112
  t/7793 -> concatenate60/113
  t/7794 -> concatenate60/114
  t/7795 -> concatenate60/115
  t/7796 -> concatenate60/116
  t/7797 -> concatenate60/117
  t/7798 -> concatenate60/118
  t/7799 -> concatenate60/119
  t/7800 -> concatenate60/120
  t/7801 -> concatenate60/121
  t/7802 -> concatenate60/122
  t/7803 -> concatenate60/123
  t/7804 -> concatenate60/124
  t/7805 -> concatenate60/125
  t/7806 -> concatenate60/126
  t/7807 -> concatenate60/127
  t/7808 -> concatenate60/128
  t/7809 -> concatenate61/1
  t/7810 -> concatenate61/2
  t/7811 -> concatenate61/3
  t/7812 -> concatenate61/4
  t/7813 -> concatenate61/5
  t/7814 -> concatenate61/6
  t/7815 -> concatenate61/7
  t/7816 -> concatenate61/8
  t/7817 -> concatenate61/9
  t/7818 -> concatenate61/10
  t/7819 -> concatenate61/11
  t/7820 -> concatenate61/12
  t/7821 -> concatenate61/13
  t/7822 -> concatenate61/14
  t/7823 -> concatenate61/15
  t/7824 -> concatenate61/16
  t/7825 -> concatenate61/17
  t/7826 -> concatenate61/18
  t/7827 -> concatenate61/19
  t/7828 -> concatenate61/20
  t/7829 -> concatenate61/21
  t/7830 -> concatenate61/22
  t/7831 -> concatenate61/23
  t/7832 -> concatenate61/24
  t/7833 -> concatenate61/25
  t/7834 -> concatenate61/26
  t/7835 -> concatenate61/27
  t/7836 -> concatenate61/28
  t/7837 -> concatenate61/29
  t/7838 -> concatenate61/30
  t/7839 -> concatenate61/31
  t/7840 -> concatenate61/32
  t/7841 -> concatenate61/33
  t/7842 -> concatenate61/34
  t/7843 -> concatenate61/35
  t/7844 -> concatenate61/36
  t/7845 -> concatenate61/37
  t/7846 -> concatenate61/38
  t/7847 -> concatenate61/39
  t/7848 -> concatenate61/40
  t/7849 -> concatenate61/41
  t/7850 -> concatenate61/42
  t/7851 -> concatenate61/43
  t/7852 -> concatenate61/44
  t/7853 -> concatenate61/45
  t/7854 -> concatenate61/46
  t/7855 -> concatenate61/47
  t/7856 -> concatenate61/48
  t/7857 -> concatenate61/49
  t/7858 -> concatenate61/50
  t/7859 -> concatenate61/51
  t/7860 -> concatenate61/52
  t/7861 -> concatenate61/53
  t/7862 -> concatenate61/54
  t/7863 -> concatenate61/55
  t/7864 -> concatenate61/56
  t/7865 -> concatenate61/57
  t/7866 -> concatenate61/58
  t/7867 -> concatenate61/59
  t/7868 -> concatenate61/60
  t/7869 -> concatenate61/61
  t/7870 -> concatenate61/62
  t/7871 -> concatenate61/63
  t/7872 -> concatenate61/64
  t/7873 -> concatenate61/65
  t/7874 -> concatenate61/66
  t/7875 -> concatenate61/67
  t/7876 -> concatenate61/68
  t/7877 -> concatenate61/69
  t/7878 -> concatenate61/70
  t/7879 -> concatenate61/71
  t/7880 -> concatenate61/72
  t/7881 -> concatenate61/73
  t/7882 -> concatenate61/74
  t/7883 -> concatenate61/75
  t/7884 -> concatenate61/76
  t/7885 -> concatenate61/77
  t/7886 -> concatenate61/78
  t/7887 -> concatenate61/79
  t/7888 -> concatenate61/80
  t/7889 -> concatenate61/81
  t/7890 -> concatenate61/82
  t/7891 -> concatenate61/83
  t/7892 -> concatenate61/84
  t/7893 -> concatenate61/85
  t/7894 -> concatenate61/86
  t/7895 -> concatenate61/87
  t/7896 -> concatenate61/88
  t/7897 -> concatenate61/89
  t/7898 -> concatenate61/90
  t/7899 -> concatenate61/91
  t/7900 -> concatenate61/92
  t/7901 -> concatenate61/93
  t/7902 -> concatenate61/94
  t/7903 -> concatenate61/95
  t/7904 -> concatenate61/96
  t/7905 -> concatenate61/97
  t/7906 -> concatenate61/98
  t/7907 -> concatenate61/99
  t/7908 -> concatenate61/100
  t/7909 -> concatenate61/101
  t/7910 -> concatenate61/102
  t/7911 -> concatenate61/103
  t/7912 -> concatenate61/104
  t/7913 -> concatenate61/105
  t/7914 -> concatenate61/106
  t/7915 -> concatenate61/107
  t/7916 -> concatenate61/108
  t/7917 -> concatenate61/109
  t/7918 -> concatenate61/110
  t/7919 -> concatenate61/111
  t/7920 -> concatenate61/112
  t/7921 -> concatenate61/113
  t/7922 -> concatenate61/114
  t/7923 -> concatenate61/115
  t/7924 -> concatenate61/116
  t/7925 -> concatenate61/117
  t/7926 -> concatenate61/118
  t/7927 -> concatenate61/119
  t/7928 -> concatenate61/120
  t/7929 -> concatenate61/121
  t/7930 -> concatenate61/122
  t/7931 -> concatenate61/123
  t/7932 -> concatenate61/124
  t/7933 -> concatenate61/125
  t/7934 -> concatenate61/126
  t/7935 -> concatenate61/127
  t/7936 -> concatenate61/128
  t/7937 -> concatenate62/1
  t/7938 -> concatenate62/2
  t/7939 -> concatenate62/3
  t/7940 -> concatenate62/4
  t/7941 -> concatenate62/5
  t/7942 -> concatenate62/6
  t/7943 -> concatenate62/7
  t/7944 -> concatenate62/8
  t/7945 -> concatenate62/9
  t/7946 -> concatenate62/10
  t/7947 -> concatenate62/11
  t/7948 -> concatenate62/12
  t/7949 -> concatenate62/13
  t/7950 -> concatenate62/14
  t/7951 -> concatenate62/15
  t/7952 -> concatenate62/16
  t/7953 -> concatenate62/17
  t/7954 -> concatenate62/18
  t/7955 -> concatenate62/19
  t/7956 -> concatenate62/20
  t/7957 -> concatenate62/21
  t/7958 -> concatenate62/22
  t/7959 -> concatenate62/23
  t/7960 -> concatenate62/24
  t/7961 -> concatenate62/25
  t/7962 -> concatenate62/26
  t/7963 -> concatenate62/27
  t/7964 -> concatenate62/28
  t/7965 -> concatenate62/29
  t/7966 -> concatenate62/30
  t/7967 -> concatenate62/31
  t/7968 -> concatenate62/32
  t/7969 -> concatenate62/33
  t/7970 -> concatenate62/34
  t/7971 -> concatenate62/35
  t/7972 -> concatenate62/36
  t/7973 -> concatenate62/37
  t/7974 -> concatenate62/38
  t/7975 -> concatenate62/39
  t/7976 -> concatenate62/40
  t/7977 -> concatenate62/41
  t/7978 -> concatenate62/42
  t/7979 -> concatenate62/43
  t/7980 -> concatenate62/44
  t/7981 -> concatenate62/45
  t/7982 -> concatenate62/46
  t/7983 -> concatenate62/47
  t/7984 -> concatenate62/48
  t/7985 -> concatenate62/49
  t/7986 -> concatenate62/50
  t/7987 -> concatenate62/51
  t/7988 -> concatenate62/52
  t/7989 -> concatenate62/53
  t/7990 -> concatenate62/54
  t/7991 -> concatenate62/55
  t/7992 -> concatenate62/56
  t/7993 -> concatenate62/57
  t/7994 -> concatenate62/58
  t/7995 -> concatenate62/59
  t/7996 -> concatenate62/60
  t/7997 -> concatenate62/61
  t/7998 -> concatenate62/62
  t/7999 -> concatenate62/63
  t/8000 -> concatenate62/64
  t/8001 -> concatenate62/65
  t/8002 -> concatenate62/66
  t/8003 -> concatenate62/67
  t/8004 -> concatenate62/68
  t/8005 -> concatenate62/69
  t/8006 -> concatenate62/70
  t/8007 -> concatenate62/71
  t/8008 -> concatenate62/72
  t/8009 -> concatenate62/73
  t/8010 -> concatenate62/74
  t/8011 -> concatenate62/75
  t/8012 -> concatenate62/76
  t/8013 -> concatenate62/77
  t/8014 -> concatenate62/78
  t/8015 -> concatenate62/79
  t/8016 -> concatenate62/80
  t/8017 -> concatenate62/81
  t/8018 -> concatenate62/82
  t/8019 -> concatenate62/83
  t/8020 -> concatenate62/84
  t/8021 -> concatenate62/85
  t/8022 -> concatenate62/86
  t/8023 -> concatenate62/87
  t/8024 -> concatenate62/88
  t/8025 -> concatenate62/89
  t/8026 -> concatenate62/90
  t/8027 -> concatenate62/91
  t/8028 -> concatenate62/92
  t/8029 -> concatenate62/93
  t/8030 -> concatenate62/94
  t/8031 -> concatenate62/95
  t/8032 -> concatenate62/96
  t/8033 -> concatenate62/97
  t/8034 -> concatenate62/98
  t/8035 -> concatenate62/99
  t/8036 -> concatenate62/100
  t/8037 -> concatenate62/101
  t/8038 -> concatenate62/102
  t/8039 -> concatenate62/103
  t/8040 -> concatenate62/104
  t/8041 -> concatenate62/105
  t/8042 -> concatenate62/106
  t/8043 -> concatenate62/107
  t/8044 -> concatenate62/108
  t/8045 -> concatenate62/109
  t/8046 -> concatenate62/110
  t/8047 -> concatenate62/111
  t/8048 -> concatenate62/112
  t/8049 -> concatenate62/113
  t/8050 -> concatenate62/114
  t/8051 -> concatenate62/115
  t/8052 -> concatenate62/116
  t/8053 -> concatenate62/117
  t/8054 -> concatenate62/118
  t/8055 -> concatenate62/119
  t/8056 -> concatenate62/120
  t/8057 -> concatenate62/121
  t/8058 -> concatenate62/122
  t/8059 -> concatenate62/123
  t/8060 -> concatenate62/124
  t/8061 -> concatenate62/125
  t/8062 -> concatenate62/126
  t/8063 -> concatenate62/127
  t/8064 -> concatenate62/128
  t/8065 -> concatenate63/1
  t/8066 -> concatenate63/2
  t/8067 -> concatenate63/3
  t/8068 -> concatenate63/4
  t/8069 -> concatenate63/5
  t/8070 -> concatenate63/6
  t/8071 -> concatenate63/7
  t/8072 -> concatenate63/8
  t/8073 -> concatenate63/9
  t/8074 -> concatenate63/10
  t/8075 -> concatenate63/11
  t/8076 -> concatenate63/12
  t/8077 -> concatenate63/13
  t/8078 -> concatenate63/14
  t/8079 -> concatenate63/15
  t/8080 -> concatenate63/16
  t/8081 -> concatenate63/17
  t/8082 -> concatenate63/18
  t/8083 -> concatenate63/19
  t/8084 -> concatenate63/20
  t/8085 -> concatenate63/21
  t/8086 -> concatenate63/22
  t/8087 -> concatenate63/23
  t/8088 -> concatenate63/24
  t/8089 -> concatenate63/25
  t/8090 -> concatenate63/26
  t/8091 -> concatenate63/27
  t/8092 -> concatenate63/28
  t/8093 -> concatenate63/29
  t/8094 -> concatenate63/30
  t/8095 -> concatenate63/31
  t/8096 -> concatenate63/32
  t/8097 -> concatenate63/33
  t/8098 -> concatenate63/34
  t/8099 -> concatenate63/35
  t/8100 -> concatenate63/36
  t/8101 -> concatenate63/37
  t/8102 -> concatenate63/38
  t/8103 -> concatenate63/39
  t/8104 -> concatenate63/40
  t/8105 -> concatenate63/41
  t/8106 -> concatenate63/42
  t/8107 -> concatenate63/43
  t/8108 -> concatenate63/44
  t/8109 -> concatenate63/45
  t/8110 -> concatenate63/46
  t/8111 -> concatenate63/47
  t/8112 -> concatenate63/48
  t/8113 -> concatenate63/49
  t/8114 -> concatenate63/50
  t/8115 -> concatenate63/51
  t/8116 -> concatenate63/52
  t/8117 -> concatenate63/53
  t/8118 -> concatenate63/54
  t/8119 -> concatenate63/55
  t/8120 -> concatenate63/56
  t/8121 -> concatenate63/57
  t/8122 -> concatenate63/58
  t/8123 -> concatenate63/59
  t/8124 -> concatenate63/60
  t/8125 -> concatenate63/61
  t/8126 -> concatenate63/62
  t/8127 -> concatenate63/63
  t/8128 -> concatenate63/64
  t/8129 -> concatenate63/65
  t/8130 -> concatenate63/66
  t/8131 -> concatenate63/67
  t/8132 -> concatenate63/68
  t/8133 -> concatenate63/69
  t/8134 -> concatenate63/70
  t/8135 -> concatenate63/71
  t/8136 -> concatenate63/72
  t/8137 -> concatenate63/73
  t/8138 -> concatenate63/74
  t/8139 -> concatenate63/75
  t/8140 -> concatenate63/76
  t/8141 -> concatenate63/77
  t/8142 -> concatenate63/78
  t/8143 -> concatenate63/79
  t/8144 -> concatenate63/80
  t/8145 -> concatenate63/81
  t/8146 -> concatenate63/82
  t/8147 -> concatenate63/83
  t/8148 -> concatenate63/84
  t/8149 -> concatenate63/85
  t/8150 -> concatenate63/86
  t/8151 -> concatenate63/87
  t/8152 -> concatenate63/88
  t/8153 -> concatenate63/89
  t/8154 -> concatenate63/90
  t/8155 -> concatenate63/91
  t/8156 -> concatenate63/92
  t/8157 -> concatenate63/93
  t/8158 -> concatenate63/94
  t/8159 -> concatenate63/95
  t/8160 -> concatenate63/96
  t/8161 -> concatenate63/97
  t/8162 -> concatenate63/98
  t/8163 -> concatenate63/99
  t/8164 -> concatenate63/100
  t/8165 -> concatenate63/101
  t/8166 -> concatenate63/102
  t/8167 -> concatenate63/103
  t/8168 -> concatenate63/104
  t/8169 -> concatenate63/105
  t/8170 -> concatenate63/106
  t/8171 -> concatenate63/107
  t/8172 -> concatenate63/108
  t/8173 -> concatenate63/109
  t/8174 -> concatenate63/110
  t/8175 -> concatenate63/111
  t/8176 -> concatenate63/112
  t/8177 -> concatenate63/113
  t/8178 -> concatenate63/114
  t/8179 -> concatenate63/115
  t/8180 -> concatenate63/116
  t/8181 -> concatenate63/117
  t/8182 -> concatenate63/118
  t/8183 -> concatenate63/119
  t/8184 -> concatenate63/120
  t/8185 -> concatenate63/121
  t/8186 -> concatenate63/122
  t/8187 -> concatenate63/123
  t/8188 -> concatenate63/124
  t/8189 -> concatenate63/125
  t/8190 -> concatenate63/126
  t/8191 -> concatenate63/127
  t/8192 -> concatenate63/128
  concatenate/1 -> concatenate64/1
  concatenate1/1 -> concatenate64/2
  concatenate2/1 -> concatenate64/3
  concatenate3/1 -> concatenate64/4
  concatenate4/1 -> concatenate64/5
  concatenate5/1 -> concatenate64/6
  concatenate6/1 -> concatenate64/7
  concatenate7/1 -> concatenate64/8
  concatenate8/1 -> concatenate64/9
  concatenate9/1 -> concatenate64/10
  concatenate10/1 -> concatenate64/11
  concatenate11/1 -> concatenate64/12
  concatenate12/1 -> concatenate64/13
  concatenate13/1 -> concatenate64/14
  concatenate14/1 -> concatenate64/15
  concatenate15/1 -> concatenate64/16
  concatenate16/1 -> concatenate64/17
  concatenate17/1 -> concatenate64/18
  concatenate18/1 -> concatenate64/19
  concatenate19/1 -> concatenate64/20
  concatenate20/1 -> concatenate64/21
  concatenate21/1 -> concatenate64/22
  concatenate22/1 -> concatenate64/23
  concatenate23/1 -> concatenate64/24
  concatenate24/1 -> concatenate64/25
  concatenate25/1 -> concatenate64/26
  concatenate26/1 -> concatenate64/27
  concatenate27/1 -> concatenate64/28
  concatenate28/1 -> concatenate64/29
  concatenate29/1 -> concatenate64/30
  concatenate30/1 -> concatenate64/31
  concatenate31/1 -> concatenate64/32
  concatenate32/1 -> concatenate64/33
  concatenate33/1 -> concatenate64/34
  concatenate34/1 -> concatenate64/35
  concatenate35/1 -> concatenate64/36
  concatenate36/1 -> concatenate64/37
  concatenate37/1 -> concatenate64/38
  concatenate38/1 -> concatenate64/39
  concatenate39/1 -> concatenate64/40
  concatenate40/1 -> concatenate64/41
  concatenate41/1 -> concatenate64/42
  concatenate42/1 -> concatenate64/43
  concatenate43/1 -> concatenate64/44
  concatenate44/1 -> concatenate64/45
  concatenate45/1 -> concatenate64/46
  concatenate46/1 -> concatenate64/47
  concatenate47/1 -> concatenate64/48
  concatenate48/1 -> concatenate64/49
  concatenate49/1 -> concatenate64/50
  concatenate50/1 -> concatenate64/51
  concatenate51/1 -> concatenate64/52
  concatenate52/1 -> concatenate64/53
  concatenate53/1 -> concatenate64/54
  concatenate54/1 -> concatenate64/55
  concatenate55/1 -> concatenate64/56
  concatenate56/1 -> concatenate64/57
  concatenate57/1 -> concatenate64/58
  concatenate58/1 -> concatenate64/59
  concatenate59/1 -> concatenate64/60
  concatenate60/1 -> concatenate64/61
  concatenate61/1 -> concatenate64/62
  concatenate62/1 -> concatenate64/63
  concatenate63/1 -> concatenate64/64
